simulink library "AEMS_Standard_Library"  (R2016b)
(part 5 of 39)

      |         else
      |             blocks_size = length(NewStatusstr);
      |             for r=length(NewStatusstr)+1:length(OldStatusstr)
      |                 lh = get_param([libb,'/Conversion_Subsystem_',num2str(r)],'Handle');
      |                 lc = get_param([libb,'/Data_Type_Conversion_',num2str(r)],'Handle');
      |                 l = get_param([libb,'/',OldStatusstr(r).Name],'Handle');
      |                 delete_block(lh);
      |                 delete_block(lc);
      |                 delete_block(l);
      |             end
      |             delete_line(find_system(libb,'FollowLinks','on','FindAll','on','LookUnderMasks','on','Type','line','Connected','off'));
      |         end
      |     end
      |     
      |     
      |     
      |     for i=1:count_DID
      |         n = num2str(i);
      |         if i==1
      |             tmp_sub = conv_subs;
      |             tmp_dataconv = data_converter;
      |             nameblk='Conversion_Subsystem';
      |         else
      |             tmp_sub = [conv_subs,'_',n];
      |             tmp_dataconv = [data_converter,'_',n];
      |             nameblk=['Conversion_Subsystem','_',n];
      |         end
      |         pos_i = get_param(tmp_sub,'Position');
      |         conv_type = get_param(tmp_sub,'MaskType');
      |         dc = get_param(tmp_dataconv,'Position');
      |         pos_i_o=pos_i;
      |         dc1 = dc;
      |         if length(upd_dmux.Outport)>=i
      |             r_upd_dmux = get(upd_dmux.Outport(i),'Position');
      |             pos_i_o(2)=r_upd_dmux(2)-(pos_i(4)-pos_i(2))/2;
      |             pos_i_o(4)=r_upd_dmux(2)+(pos_i(4)-pos_i(2))/2;
      |             dc1(2) = r_upd_dmux(2)-(dc(4)-dc(2))/2;
      |             dc1(4) = r_upd_dmux(2)+(dc(4)-dc(2))/2;
      |         end
      |         set_param(tmp_sub,'Position',pos_i_o);
      |         set_param(tmp_dataconv,'Position',dc1);
      |         
      |         ph_h = get_param(tmp_sub,'PortHandles');
      |         add_line(libb,ph_dmux.Outport(i),ph_h.Inport,'Autorouting','On');
      |         set_param(tmp_sub,'ShowName','off');
      |         set_param(tmp_dataconv,'ShowName','off');
      |         if ismember(NewStatusstr(i).DID_DataType,{'uint8','int8'}) && ~strcmp(conv_type,'AEMS_CONVERT_BYTE_TO_FLP')
      |             %If the ctrl reaches here means, this did is changed from Multibyte to 1 byte.
      |             replace_block(libb,'FollowLinks', 'on','Name',nameblk,'AEMS_Standard_Library/SUB/AEMS_CONVERT_BYTE_TO_FLP','noprompt');
      |         elseif ~ismember(NewStatusstr(i).DID_DataType,{'uint8','int8'}) && strcmp(conv_type,'AEMS_CONVERT_BYTE_TO_FLP')
      |             replace_block(libb,'FollowLinks', 'on','Name',nameblk,'AEMS_Standard_Library/SUB/AEMS_CONVERT_BUFFER_TO_FLP','noprompt');
      |         end
      |         set_param(tmp_sub,...
      |             'Resol',NewStatusstr(i).Resol,...
      |             'offset',NewStatusstr(i).Offset,...
      |             'DID_Datatype',NewStatusstr(i).DID_DataType);
      |         convertblk=get_param(tmp_sub,'LineHandles');
      |         datacovblk=get_param(tmp_dataconv,'LineHandles');
      |         dstblkhdl=get_param(datacovblk.Outport,'DstBlockHandle');
      |         if dstblkhdl==1
      |             ports_name = dstblkhdl;
      |         elseif dstblkhdl > 1
      |             if isequal(get_param(dstblkhdl(1),'BlockType'),'Outport')
      |                 ports_name = dstblkhdl(1);
      |             elseif isequal(get_param(dstblkhdl(2),'BlockType'),'Outport')
      |                 ports_name = dstblkhdl(2);
      |             end
      |         end
      |         
      |         set_param(ports_name,'Name',NewStatusstr(i).Name);
      |         pos_out_i = get_param(ports_name,'Position');
      |         
      |         pos_out_i_o=pos_out_i;
      |         pos_out_i_o(2)=(pos_i_o(2)+pos_i_o(4))/2-(pos_out_i(4)-pos_out_i(2))/2;
      |         pos_out_i_o(4)=(pos_i_o(2)+pos_i_o(4))/2+(pos_out_i(4)-pos_out_i(2))/2;
      |         set_param(dstblkhdl(1),'Position',pos_out_i_o);
      |     end
      | end
      | for i=1:blocks_size
      |     if i==1
      |         conv_blk_name = [libb,'/Conversion_Subsystem'];
      |     else
      |         conv_blk_name = [libb,'/Conversion_Subsystem_',num2str(i)];
      |     end
      |     if ~isequal(NewStatusstr(i).DID_DataType,OldStatusstr(i).DID_DataType)
      |         name_blk = get_param(conv_blk_name,'Name');
      |         if ismember(NewStatusstr(i).DID_DataType,{'uint8','int8'}) && ~ismember(OldStatusstr(i).DID_DataType,{'uint8','int8'})
      |             replace_block(libb,'FollowLinks', 'on','Name',name_blk,'AEMS_Standard_Library/SUB/AEMS_CONVERT_BYTE_TO_FLP','noprompt');
      |         elseif ~ismember(NewStatusstr(i).DID_DataType,{'uint8','int8'}) && ismember(OldStatusstr(i).DID_DataType,{'uint8','int8'})
      |             replace_block(libb,'FollowLinks', 'on','Name',name_blk,'AEMS_Standard_Library/SUB/AEMS_CONVERT_BUFFER_TO_FLP','noprompt');
      |         end
      |         set_param(conv_blk_name,'DID_Datatype',NewStatusstr(i).DID_DataType);
      |     end
      |     if ~isequal(NewStatusstr(i).Resol,OldStatusstr(i).Resol)
      |         set_param(conv_blk_name,'Resol',NewStatusstr(i).Resol);
      |     end
      |     if ~isequal(NewStatusstr(i).Offset,OldStatusstr(i).Offset)
      |         set_param(conv_blk_name,'offset',NewStatusstr(i).Offset);
      |     end
      |     if ~isequal(NewStatusstr(i).Name,OldStatusstr(i).Name)&& ~chg_status
      |         set(ou{i},'Name',NewStatusstr(i).Name);
      |     end
      | end
      | txtvisibility='%<MaskType> \n ConfigManagement : %<ConfigManagement> \n DID Abstract: %<DIDAbstract> \n Number of DID Variables: %<NumDIDVar>';
      | for i=1:count_DID
      |     n = num2str(i);
      |     txtvisibility=[txtvisibility,'\n %<OutVarName_',n,'> : {Resol = %<ResolDID_',n,'>, Offset = %<OffsetDID_',n,'>, DID_Monitoring_DataType = %<DataType_DID_',n,'>}'];
      | end
      | % wrfly_old = find_system(libh,'FollowLinks','on','LookunderMasks','all','MaskType','AEMS_NVM_WRITEONFLY');
      | % wrfly_new = get(libh,'NVMChecked');
      | % N_Inports=get_param(libb,'NumDIDVar');
      | % if strcmp(wrfly_new,'off')
      | %     if ~isempty(wrfly_old)
      | %         lh_wr = get_param(wr_fly,'LineHandles');
      | %         for hdl_len = 1:length(lh_wr.Inport)
      | %             if lh_wr.Inport(hdl_len)>0
      | %                 delete_line(lh_wr.Inport(hdl_len));
      | %             end
      | %         end
      | %         delete_line(lh_wr.Enable);
      | %         delete_block(wr_fly);
      | %     end
      | %     txtvisibility=[txtvisibility,'\n NVM WriteOnFly Variables : %<NVMChecked>'];
      | % else
      | %     if isempty(wrfly_old)
      | %         call_sub = get_param([libb,'/Callback_Subsystem'],'Position');
      | %         wrf_hand = add_block('AEMS_Standard_Library/MEM/AEMS_NVM_WRITEONFLY',[libb,'/AEMS_NVM_WRITEONFLY'],...
      | %             'Position',[call_sub(1)-200 call_sub(4)+50 call_sub(1)+50 call_sub(4)+120],'ChId',get_param(libb,'Channel'),'TriggerType','Enable');
      | %         lh_wr = get_param(wrf_hand,'PortHandles');
      | %         lh_perm = get_param(perm_sub,'PortHandles');
      | %         add_line(libb,lh_perm.Outport,lh_wr.Enable,'Autorouting','On');
      | %     else
      | %         newnvmchannel=get_param(libb,'Channel');
      | %         oldnvmchannel=get_param(wrfly_old,'ChId');
      | %         if ~strcmpi(newnvmchannel,oldnvmchannel)
      | %             set_param(wrfly_old,'ChId',newnvmchannel);
      | %         end
      | %     end
      | %     if isempty(wrfly_old)|| chg_status
      | %         write_hdles = get_param([libb,'/AEMS_NVM_WRITEONFLY'],'LineHandles');
      | %         for hdl_len = 1:length(write_hdles.Inport)
      | %             if ~isequal(write_hdles.Inport(hdl_len),-1)
      | %                 delete_line(write_hdles.Inport(hdl_len));
      | %             end
      | %         end
      | %         set_param([libb,'/AEMS_NVM_WRITEONFLY'],'NumInputs',N_Inports);
      | %         write_port = get_param([libb,'/AEMS_NVM_WRITEONFLY'],'PortHandles');
      | %         for r=1:length(NewStatusstr)
      | %             if(r==1)
      | %                 conversion_hdl = get_param([libb,'/Data_Type_Conversion'],'PortHandles');
      | %             else
      | %                 conversion_hdl = get_param([libb,'/Data_Type_Conversion_',num2str(r)],'PortHandles');
      | %             end
      | %             add_line(libb,conversion_hdl.Outport,write_port.Inport(r),'Autorouting','On');
      | %         end
      | %     end
      | %     txtvisibility=[txtvisibility,'\n NVM WriteOnFly Variables : %<NVMChecked> \n WriteOnFly Channel : %<Channel>'];
      | % end
      | % if ~strcmp(txtvisibility,old_txtvisibility)
      | %     set(libh,'AttributesFormatString',txtvisibility);
      | % end
      settings: AttributesFormatString=%<MaskType> \n ConfigManagement : %<ConfigManagement> \n DID Abstract: %<DIDAbstract> \n Number of DID Variables: %<NumDIDVar>\n %<OutVarName_1> : {Resol = %<ResolDID_1>, Offset = %<OffsetDID_1>, DID_Monitoring_DataType = %<DataType_DID_1>}
      mask Help:
      | eval('path_lib=fileparts(which(''AEMS_Standard_Library''));');
      | doc_path = [path_lib '\help\AEMS_DCM_DID_WRITEDATA.pdf'];
      | eval('open(doc_path)')
      mask TypeOptions NumDIDVar: 1 | 2 | 3 | 4 | 5 | 6 | 7 | 8 | 9 | 10 | 11 | 12 | 13 | 14 | 15 | 16 | 17 | 18 | 19 | 20 | 21 | 22 | 23 | 24 | 25 | 26 | 27 | 28 | 29 | 30 | 31 | 32 | 33 | 34 | 35 | 36 | 37 | 38 | 39 | 40 | 41 | 42 | 43 | 44 | 45 | 46 | 47 | 48 | 49 | 50 | 51 | 52 | 53 | 54 | 55 | 56 | 57 | 58 | 59 | 60 | 61 | 62 | 63 | 64 | 65 | 66 | 67 | 68 | 69 | 70 | 71 | 72 | 73 | 74 | 75 | 76 | 77 | 78 | 79 | 80 | 81 | 82 | 83 | 84 | 85 | 86 | 87 | 88 | 89 | 90 | 91 | 92 | 93 | 94 | 95 | 96 | 97 | 98 | 99 | 100 | 101 | 102 | 103 | 104 | 105 | 106 | 107 | 108 | 109 | 110 | 111 | 112 | 113 | 114 | 115 | 116 | 117 | 118 | 119 | 120 | 121 | 122 | 123 | 124 | 125 | 126 | 127 | 128 | 129 | 130 | 131 | 132 | 133 | 134 | 135 | 136 | 137 | 138 | 139 | 140 | 141 | 142 | 143 | 144 | 145 | 146 | 147 | 148 | 149 | 150 | 151 | 152 | 153 | 154 | 155 | 156 | 157 | 158 | 159 | 160 | 161 | 162 | 163 | 164 | 165 | 166 | 167 | 168 | 169 | 170 | 171 | 172 | 173 | 174 | 175 | 176 | 177 | 178 | 179 | 180 | 181 | 182 | 183 | 184 | 185 | 186 | 187 | 188 | 189 | 190 | 191 | 192 | 193 | 194 | 195 | 196 | 197 | 198 | 199 | 200 | 201 | 202 | 203 | 204 | 205 | 206 | 207 | 208 | 209 | 210 | 211 | 212 | 213 | 214 | 215 | 216 | 217 | 218 | 219 | 220 | 221 | 222 | 223 | 224 | 225 | 226 | 227 | 228 | 229 | 230 | 231 | 232 | 233 | 234 | 235 | 236 | 237 | 238 | 239 | 240 | 241 | 242 | 243 | 244 | 245 | 246 | 247 | 248 | 249 | 250 | 251 | 252 | 253 | 254 | 255 | 256 | 257 | 258 | 259 | 260 | 261 | 262 | 263 | 264 | 265 | 266 | 267 | 268 | 269 | 270 | 271 | 272 | 273 | 274 | 275 | 276 | 277 | 278 | 279 | 280 | 281 | 282 | 283 | 284 | 285 | 286 | 287 | 288 | 289 | 290 | 291 | 292 | 293 | 294 | 295 | 296 | 297 | 298 | 299 | 300 | 301 | 302 | 303 | 304 | 305 | 306 | 307 | 308 | 309 | 310 | 311 | 312 | 313 | 314 | 315 | 316 | 317 | 318 | 319 | 320 | 321 | 322 | 323 | 324 | 325 | 326 | 327 | 328 | 329 | 330 | 331 | 332 | 333 | 334 | 335 | 336 | 337 | 338 | 339 | 340 | 341 | 342 | 343 | 344 | 345 | 346 | 347 | 348 | 349 | 350 | 351 | 352 | 353 | 354 | 355 | 356 | 357 | 358 | 359 | 360 | 361 | 362 | 363 | 364 | 365 | 366 | 367 | 368 | 369 | 370 | 371 | 372 | 373 | 374 | 375 | 376 | 377 | 378 | 379 | 380 | 381 | 382 | 383 | 384 | 385 | 386 | 387 | 388 | 389 | 390 | 391 | 392 | 393 | 394 | 395 | 396 | 397 | 398 | 399 | 400
      mask Callback NumDIDVar:
      | DCM_WR_DATA_NumDIDVar = str2double(get(gcbh,'NumDIDVar'));
      | maskobj = Simulink.Mask.get(gcbh);
      | maskobj_old = maskobj.getDialogControls();
      | DCM_WR_DATA_second = maskobj_old.DialogControls(2);
      | show_hide_DID = DCM_WR_DATA_second.DialogControls;
      | 
      | for DID_j=2:length(show_hide_DID)
      |     show_hide_DID(DID_j).Visible = 'off';
      | end
      | 
      | for DID_j=DCM_WR_DATA_NumDIDVar+1:-1:2
      |     show_hide_DID(DID_j).Visible = 'on';
      | end
      | 
      | clear DCM_WR_DATA_NumDIDVar;
      | clear show_hide_DID;
      | clear maskobj;
      | clear maskobj_old;
      | clear DID_j;
      | clear DCM_WR_DATA_second;
      mask TypeOptions DataType_DID_1: int8 | uint8 | int16 | uint16 | int32 | uint32
      mask TypeOptions DataType_DID_2: int8 | uint8 | int16 | uint16 | int32 | uint32
      mask TypeOptions DataType_DID_3: int8 | uint8 | int16 | uint16 | int32 | uint32
      mask TypeOptions DataType_DID_4: int8 | uint8 | int16 | uint16 | int32 | uint32
      mask TypeOptions DataType_DID_5: int8 | uint8 | int16 | uint16 | int32 | uint32
      mask TypeOptions DataType_DID_6: int8 | uint8 | int16 | uint16 | int32 | uint32
      mask TypeOptions DataType_DID_7: int8 | uint8 | int16 | uint16 | int32 | uint32
      mask TypeOptions DataType_DID_8: int8 | uint8 | int16 | uint16 | int32 | uint32
      mask TypeOptions DataType_DID_9: int8 | uint8 | int16 | uint16 | int32 | uint32
      mask TypeOptions DataType_DID_10: int8 | uint8 | int16 | uint16 | int32 | uint32
      mask TypeOptions DataType_DID_11: int8 | uint8 | int16 | uint16 | int32 | uint32
      mask TypeOptions DataType_DID_12: int8 | uint8 | int16 | uint16 | int32 | uint32
      mask TypeOptions DataType_DID_13: int8 | uint8 | int16 | uint16 | int32 | uint32
      mask TypeOptions DataType_DID_14: int8 | uint8 | int16 | uint16 | int32 | uint32
      mask TypeOptions DataType_DID_15: int8 | uint8 | int16 | uint16 | int32 | uint32
      mask TypeOptions DataType_DID_16: int8 | uint8 | int16 | uint16 | int32 | uint32
      mask TypeOptions DataType_DID_17: int8 | uint8 | int16 | uint16 | int32 | uint32
      mask TypeOptions DataType_DID_18: int8 | uint8 | int16 | uint16 | int32 | uint32
      mask TypeOptions DataType_DID_19: int8 | uint8 | int16 | uint16 | int32 | uint32
      mask TypeOptions DataType_DID_20: int8 | uint8 | int16 | uint16 | int32 | uint32
      mask TypeOptions DataType_DID_21: int8 | uint8 | int16 | uint16 | int32 | uint32
      mask TypeOptions DataType_DID_22: int8 | uint8 | int16 | uint16 | int32 | uint32
      mask TypeOptions DataType_DID_23: int8 | uint8 | int16 | uint16 | int32 | uint32
      mask TypeOptions DataType_DID_24: int8 | uint8 | int16 | uint16 | int32 | uint32
      mask TypeOptions DataType_DID_25: int8 | uint8 | int16 | uint16 | int32 | uint32
      mask TypeOptions DataType_DID_26: int8 | uint8 | int16 | uint16 | int32 | uint32
      mask TypeOptions DataType_DID_27: int8 | uint8 | int16 | uint16 | int32 | uint32
      mask TypeOptions DataType_DID_28: int8 | uint8 | int16 | uint16 | int32 | uint32
      mask TypeOptions DataType_DID_29: int8 | uint8 | int16 | uint16 | int32 | uint32
      mask TypeOptions DataType_DID_30: int8 | uint8 | int16 | uint16 | int32 | uint32
      mask TypeOptions DataType_DID_31: int8 | uint8 | int16 | uint16 | int32 | uint32
      mask TypeOptions DataType_DID_32: int8 | uint8 | int16 | uint16 | int32 | uint32
      mask TypeOptions DataType_DID_33: int8 | uint8 | int16 | uint16 | int32 | uint32
      mask TypeOptions DataType_DID_34: int8 | uint8 | int16 | uint16 | int32 | uint32
      mask TypeOptions DataType_DID_35: int8 | uint8 | int16 | uint16 | int32 | uint32
      mask TypeOptions DataType_DID_36: int8 | uint8 | int16 | uint16 | int32 | uint32
      mask TypeOptions DataType_DID_37: int8 | uint8 | int16 | uint16 | int32 | uint32
      mask TypeOptions DataType_DID_38: int8 | uint8 | int16 | uint16 | int32 | uint32
      mask TypeOptions DataType_DID_39: int8 | uint8 | int16 | uint16 | int32 | uint32
      mask TypeOptions DataType_DID_40: int8 | uint8 | int16 | uint16 | int32 | uint32
      mask TypeOptions DataType_DID_41: int8 | uint8 | int16 | uint16 | int32 | uint32
      mask TypeOptions DataType_DID_42: int8 | uint8 | int16 | uint16 | int32 | uint32
      mask TypeOptions DataType_DID_43: int8 | uint8 | int16 | uint16 | int32 | uint32
      mask TypeOptions DataType_DID_44: int8 | uint8 | int16 | uint16 | int32 | uint32
      mask TypeOptions DataType_DID_45: int8 | uint8 | int16 | uint16 | int32 | uint32
      mask TypeOptions DataType_DID_46: int8 | uint8 | int16 | uint16 | int32 | uint32
      mask TypeOptions DataType_DID_47: int8 | uint8 | int16 | uint16 | int32 | uint32
      mask TypeOptions DataType_DID_48: int8 | uint8 | int16 | uint16 | int32 | uint32
      mask TypeOptions DataType_DID_49: int8 | uint8 | int16 | uint16 | int32 | uint32
      mask TypeOptions DataType_DID_50: int8 | uint8 | int16 | uint16 | int32 | uint32
      mask TypeOptions DataType_DID_51: int8 | uint8 | int16 | uint16 | int32 | uint32
      mask TypeOptions DataType_DID_52: int8 | uint8 | int16 | uint16 | int32 | uint32
      mask TypeOptions DataType_DID_53: int8 | uint8 | int16 | uint16 | int32 | uint32
      mask TypeOptions DataType_DID_54: int8 | uint8 | int16 | uint16 | int32 | uint32
      mask TypeOptions DataType_DID_55: int8 | uint8 | int16 | uint16 | int32 | uint32
      mask TypeOptions DataType_DID_56: int8 | uint8 | int16 | uint16 | int32 | uint32
      mask TypeOptions DataType_DID_57: int8 | uint8 | int16 | uint16 | int32 | uint32
      mask TypeOptions DataType_DID_58: int8 | uint8 | int16 | uint16 | int32 | uint32
      mask TypeOptions DataType_DID_59: int8 | uint8 | int16 | uint16 | int32 | uint32
      mask TypeOptions DataType_DID_60: int8 | uint8 | int16 | uint16 | int32 | uint32
      mask TypeOptions DataType_DID_61: int8 | uint8 | int16 | uint16 | int32 | uint32
      mask TypeOptions DataType_DID_62: int8 | uint8 | int16 | uint16 | int32 | uint32
      mask TypeOptions DataType_DID_63: int8 | uint8 | int16 | uint16 | int32 | uint32
      mask TypeOptions DataType_DID_64: int8 | uint8 | int16 | uint16 | int32 | uint32
      mask TypeOptions DataType_DID_65: int8 | uint8 | int16 | uint16 | int32 | uint32
      mask TypeOptions DataType_DID_66: int8 | uint8 | int16 | uint16 | int32 | uint32
      mask TypeOptions DataType_DID_67: int8 | uint8 | int16 | uint16 | int32 | uint32
      mask TypeOptions DataType_DID_68: int8 | uint8 | int16 | uint16 | int32 | uint32
      mask TypeOptions DataType_DID_69: int8 | uint8 | int16 | uint16 | int32 | uint32
      mask TypeOptions DataType_DID_70: int8 | uint8 | int16 | uint16 | int32 | uint32
      mask TypeOptions DataType_DID_71: int8 | uint8 | int16 | uint16 | int32 | uint32
      mask TypeOptions DataType_DID_72: int8 | uint8 | int16 | uint16 | int32 | uint32
      mask TypeOptions DataType_DID_73: int8 | uint8 | int16 | uint16 | int32 | uint32
      mask TypeOptions DataType_DID_74: int8 | uint8 | int16 | uint16 | int32 | uint32
      mask TypeOptions DataType_DID_75: int8 | uint8 | int16 | uint16 | int32 | uint32
      mask TypeOptions DataType_DID_76: int8 | uint8 | int16 | uint16 | int32 | uint32
      mask TypeOptions DataType_DID_77: int8 | uint8 | int16 | uint16 | int32 | uint32
      mask TypeOptions DataType_DID_78: int8 | uint8 | int16 | uint16 | int32 | uint32
      mask TypeOptions DataType_DID_79: int8 | uint8 | int16 | uint16 | int32 | uint32
      mask TypeOptions DataType_DID_80: int8 | uint8 | int16 | uint16 | int32 | uint32
      mask TypeOptions DataType_DID_81: int8 | uint8 | int16 | uint16 | int32 | uint32
      mask TypeOptions DataType_DID_82: int8 | uint8 | int16 | uint16 | int32 | uint32
      mask TypeOptions DataType_DID_83: int8 | uint8 | int16 | uint16 | int32 | uint32
      mask TypeOptions DataType_DID_84: int8 | uint8 | int16 | uint16 | int32 | uint32
      mask TypeOptions DataType_DID_85: int8 | uint8 | int16 | uint16 | int32 | uint32
      mask TypeOptions DataType_DID_86: int8 | uint8 | int16 | uint16 | int32 | uint32
      mask TypeOptions DataType_DID_87: int8 | uint8 | int16 | uint16 | int32 | uint32
      mask TypeOptions DataType_DID_88: int8 | uint8 | int16 | uint16 | int32 | uint32
      mask TypeOptions DataType_DID_89: int8 | uint8 | int16 | uint16 | int32 | uint32
      mask TypeOptions DataType_DID_90: int8 | uint8 | int16 | uint16 | int32 | uint32
      mask TypeOptions DataType_DID_91: int8 | uint8 | int16 | uint16 | int32 | uint32
      mask TypeOptions DataType_DID_92: int8 | uint8 | int16 | uint16 | int32 | uint32
      mask TypeOptions DataType_DID_93: int8 | uint8 | int16 | uint16 | int32 | uint32
      mask TypeOptions DataType_DID_94: int8 | uint8 | int16 | uint16 | int32 | uint32
      mask TypeOptions DataType_DID_95: int8 | uint8 | int16 | uint16 | int32 | uint32
      mask TypeOptions DataType_DID_96: int8 | uint8 | int16 | uint16 | int32 | uint32
      mask TypeOptions DataType_DID_97: int8 | uint8 | int16 | uint16 | int32 | uint32
      mask TypeOptions DataType_DID_98: int8 | uint8 | int16 | uint16 | int32 | uint32
      mask TypeOptions DataType_DID_99: int8 | uint8 | int16 | uint16 | int32 | uint32
      mask TypeOptions DataType_DID_100: int8 | uint8 | int16 | uint16 | int32 | uint32
      mask TypeOptions DataType_DID_101: int8 | uint8 | int16 | uint16 | int32 | uint32
      mask TypeOptions DataType_DID_102: int8 | uint8 | int16 | uint16 | int32 | uint32
      mask TypeOptions DataType_DID_103: int8 | uint8 | int16 | uint16 | int32 | uint32
      mask TypeOptions DataType_DID_104: int8 | uint8 | int16 | uint16 | int32 | uint32
      mask TypeOptions DataType_DID_105: int8 | uint8 | int16 | uint16 | int32 | uint32
      mask TypeOptions DataType_DID_106: int8 | uint8 | int16 | uint16 | int32 | uint32
      mask TypeOptions DataType_DID_107: int8 | uint8 | int16 | uint16 | int32 | uint32
      mask TypeOptions DataType_DID_108: int8 | uint8 | int16 | uint16 | int32 | uint32
      mask TypeOptions DataType_DID_109: int8 | uint8 | int16 | uint16 | int32 | uint32
      mask TypeOptions DataType_DID_110: int8 | uint8 | int16 | uint16 | int32 | uint32
      mask TypeOptions DataType_DID_111: int8 | uint8 | int16 | uint16 | int32 | uint32
      mask TypeOptions DataType_DID_112: int8 | uint8 | int16 | uint16 | int32 | uint32
      mask TypeOptions DataType_DID_113: int8 | uint8 | int16 | uint16 | int32 | uint32
      mask TypeOptions DataType_DID_114: int8 | uint8 | int16 | uint16 | int32 | uint32
      mask TypeOptions DataType_DID_115: int8 | uint8 | int16 | uint16 | int32 | uint32
      mask TypeOptions DataType_DID_116: int8 | uint8 | int16 | uint16 | int32 | uint32
      mask TypeOptions DataType_DID_117: int8 | uint8 | int16 | uint16 | int32 | uint32
      mask TypeOptions DataType_DID_118: int8 | uint8 | int16 | uint16 | int32 | uint32
      mask TypeOptions DataType_DID_119: int8 | uint8 | int16 | uint16 | int32 | uint32
      mask TypeOptions DataType_DID_120: int8 | uint8 | int16 | uint16 | int32 | uint32
      mask TypeOptions DataType_DID_121: int8 | uint8 | int16 | uint16 | int32 | uint32
      mask TypeOptions DataType_DID_122: int8 | uint8 | int16 | uint16 | int32 | uint32
      mask TypeOptions DataType_DID_123: int8 | uint8 | int16 | uint16 | int32 | uint32
      mask TypeOptions DataType_DID_124: int8 | uint8 | int16 | uint16 | int32 | uint32
      mask TypeOptions DataType_DID_125: int8 | uint8 | int16 | uint16 | int32 | uint32
      mask TypeOptions DataType_DID_126: int8 | uint8 | int16 | uint16 | int32 | uint32
      mask TypeOptions DataType_DID_127: int8 | uint8 | int16 | uint16 | int32 | uint32
      mask TypeOptions DataType_DID_128: int8 | uint8 | int16 | uint16 | int32 | uint32
      mask TypeOptions DataType_DID_129: int8 | uint8 | int16 | uint16 | int32 | uint32
      mask TypeOptions DataType_DID_130: int8 | uint8 | int16 | uint16 | int32 | uint32
      mask TypeOptions DataType_DID_131: int8 | uint8 | int16 | uint16 | int32 | uint32
      mask TypeOptions DataType_DID_132: int8 | uint8 | int16 | uint16 | int32 | uint32
      mask TypeOptions DataType_DID_133: int8 | uint8 | int16 | uint16 | int32 | uint32
      mask TypeOptions DataType_DID_134: int8 | uint8 | int16 | uint16 | int32 | uint32
      mask TypeOptions DataType_DID_135: int8 | uint8 | int16 | uint16 | int32 | uint32
      mask TypeOptions DataType_DID_136: int8 | uint8 | int16 | uint16 | int32 | uint32
      mask TypeOptions DataType_DID_137: int8 | uint8 | int16 | uint16 | int32 | uint32
      mask TypeOptions DataType_DID_138: int8 | uint8 | int16 | uint16 | int32 | uint32
      mask TypeOptions DataType_DID_139: int8 | uint8 | int16 | uint16 | int32 | uint32
      mask TypeOptions DataType_DID_140: int8 | uint8 | int16 | uint16 | int32 | uint32
      mask TypeOptions DataType_DID_141: int8 | uint8 | int16 | uint16 | int32 | uint32
      mask TypeOptions DataType_DID_142: int8 | uint8 | int16 | uint16 | int32 | uint32
      mask TypeOptions DataType_DID_143: int8 | uint8 | int16 | uint16 | int32 | uint32
      mask TypeOptions DataType_DID_144: int8 | uint8 | int16 | uint16 | int32 | uint32
      mask TypeOptions DataType_DID_145: int8 | uint8 | int16 | uint16 | int32 | uint32
      mask TypeOptions DataType_DID_146: int8 | uint8 | int16 | uint16 | int32 | uint32
      mask TypeOptions DataType_DID_147: int8 | uint8 | int16 | uint16 | int32 | uint32
      mask TypeOptions DataType_DID_148: int8 | uint8 | int16 | uint16 | int32 | uint32
      mask TypeOptions DataType_DID_149: int8 | uint8 | int16 | uint16 | int32 | uint32
      mask TypeOptions DataType_DID_150: int8 | uint8 | int16 | uint16 | int32 | uint32
      mask TypeOptions DataType_DID_151: int8 | uint8 | int16 | uint16 | int32 | uint32
      mask TypeOptions DataType_DID_152: int8 | uint8 | int16 | uint16 | int32 | uint32
      mask TypeOptions DataType_DID_153: int8 | uint8 | int16 | uint16 | int32 | uint32
      mask TypeOptions DataType_DID_154: int8 | uint8 | int16 | uint16 | int32 | uint32
      mask TypeOptions DataType_DID_155: int8 | uint8 | int16 | uint16 | int32 | uint32
      mask TypeOptions DataType_DID_156: int8 | uint8 | int16 | uint16 | int32 | uint32
      mask TypeOptions DataType_DID_157: int8 | uint8 | int16 | uint16 | int32 | uint32
      mask TypeOptions DataType_DID_158: int8 | uint8 | int16 | uint16 | int32 | uint32
      mask TypeOptions DataType_DID_159: int8 | uint8 | int16 | uint16 | int32 | uint32
      mask TypeOptions DataType_DID_160: int8 | uint8 | int16 | uint16 | int32 | uint32
      mask TypeOptions DataType_DID_161: int8 | uint8 | int16 | uint16 | int32 | uint32
      mask TypeOptions DataType_DID_162: int8 | uint8 | int16 | uint16 | int32 | uint32
      mask TypeOptions DataType_DID_163: int8 | uint8 | int16 | uint16 | int32 | uint32
      mask TypeOptions DataType_DID_164: int8 | uint8 | int16 | uint16 | int32 | uint32
      mask TypeOptions DataType_DID_165: int8 | uint8 | int16 | uint16 | int32 | uint32
      mask TypeOptions DataType_DID_166: int8 | uint8 | int16 | uint16 | int32 | uint32
      mask TypeOptions DataType_DID_167: int8 | uint8 | int16 | uint16 | int32 | uint32
      mask TypeOptions DataType_DID_168: int8 | uint8 | int16 | uint16 | int32 | uint32
      mask TypeOptions DataType_DID_169: int8 | uint8 | int16 | uint16 | int32 | uint32
      mask TypeOptions DataType_DID_170: int8 | uint8 | int16 | uint16 | int32 | uint32
      mask TypeOptions DataType_DID_171: int8 | uint8 | int16 | uint16 | int32 | uint32
      mask TypeOptions DataType_DID_172: int8 | uint8 | int16 | uint16 | int32 | uint32
      mask TypeOptions DataType_DID_173: int8 | uint8 | int16 | uint16 | int32 | uint32
      mask TypeOptions DataType_DID_174: int8 | uint8 | int16 | uint16 | int32 | uint32
      mask TypeOptions DataType_DID_175: int8 | uint8 | int16 | uint16 | int32 | uint32
      mask TypeOptions DataType_DID_176: int8 | uint8 | int16 | uint16 | int32 | uint32
      mask TypeOptions DataType_DID_177: int8 | uint8 | int16 | uint16 | int32 | uint32
      mask TypeOptions DataType_DID_178: int8 | uint8 | int16 | uint16 | int32 | uint32
      mask TypeOptions DataType_DID_179: int8 | uint8 | int16 | uint16 | int32 | uint32
      mask TypeOptions DataType_DID_180: int8 | uint8 | int16 | uint16 | int32 | uint32
      mask TypeOptions DataType_DID_181: int8 | uint8 | int16 | uint16 | int32 | uint32
      mask TypeOptions DataType_DID_182: int8 | uint8 | int16 | uint16 | int32 | uint32
      mask TypeOptions DataType_DID_183: int8 | uint8 | int16 | uint16 | int32 | uint32
      mask TypeOptions DataType_DID_184: int8 | uint8 | int16 | uint16 | int32 | uint32
      mask TypeOptions DataType_DID_185: int8 | uint8 | int16 | uint16 | int32 | uint32
      mask TypeOptions DataType_DID_186: int8 | uint8 | int16 | uint16 | int32 | uint32
      mask TypeOptions DataType_DID_187: int8 | uint8 | int16 | uint16 | int32 | uint32
      mask TypeOptions DataType_DID_188: int8 | uint8 | int16 | uint16 | int32 | uint32
      mask TypeOptions DataType_DID_189: int8 | uint8 | int16 | uint16 | int32 | uint32
      mask TypeOptions DataType_DID_190: int8 | uint8 | int16 | uint16 | int32 | uint32
      mask TypeOptions DataType_DID_191: int8 | uint8 | int16 | uint16 | int32 | uint32
      mask TypeOptions DataType_DID_192: int8 | uint8 | int16 | uint16 | int32 | uint32
      mask TypeOptions DataType_DID_193: int8 | uint8 | int16 | uint16 | int32 | uint32
      mask TypeOptions DataType_DID_194: int8 | uint8 | int16 | uint16 | int32 | uint32
      mask TypeOptions DataType_DID_195: int8 | uint8 | int16 | uint16 | int32 | uint32
      mask TypeOptions DataType_DID_196: int8 | uint8 | int16 | uint16 | int32 | uint32
      mask TypeOptions DataType_DID_197: int8 | uint8 | int16 | uint16 | int32 | uint32
      mask TypeOptions DataType_DID_198: int8 | uint8 | int16 | uint16 | int32 | uint32
      mask TypeOptions DataType_DID_199: int8 | uint8 | int16 | uint16 | int32 | uint32
      mask TypeOptions DataType_DID_200: int8 | uint8 | int16 | uint16 | int32 | uint32
      mask TypeOptions DataType_DID_201: int8 | uint8 | int16 | uint16 | int32 | uint32
      mask TypeOptions DataType_DID_202: int8 | uint8 | int16 | uint16 | int32 | uint32
      mask TypeOptions DataType_DID_203: int8 | uint8 | int16 | uint16 | int32 | uint32
      mask TypeOptions DataType_DID_204: int8 | uint8 | int16 | uint16 | int32 | uint32
      mask TypeOptions DataType_DID_205: int8 | uint8 | int16 | uint16 | int32 | uint32
      mask TypeOptions DataType_DID_206: int8 | uint8 | int16 | uint16 | int32 | uint32
      mask TypeOptions DataType_DID_207: int8 | uint8 | int16 | uint16 | int32 | uint32
      mask TypeOptions DataType_DID_208: int8 | uint8 | int16 | uint16 | int32 | uint32
      mask TypeOptions DataType_DID_209: int8 | uint8 | int16 | uint16 | int32 | uint32
      mask TypeOptions DataType_DID_210: int8 | uint8 | int16 | uint16 | int32 | uint32
      mask TypeOptions DataType_DID_211: int8 | uint8 | int16 | uint16 | int32 | uint32
      mask TypeOptions DataType_DID_212: int8 | uint8 | int16 | uint16 | int32 | uint32
      mask TypeOptions DataType_DID_213: int8 | uint8 | int16 | uint16 | int32 | uint32
      mask TypeOptions DataType_DID_214: int8 | uint8 | int16 | uint16 | int32 | uint32
      mask TypeOptions DataType_DID_215: int8 | uint8 | int16 | uint16 | int32 | uint32
      mask TypeOptions DataType_DID_216: int8 | uint8 | int16 | uint16 | int32 | uint32
      mask TypeOptions DataType_DID_217: int8 | uint8 | int16 | uint16 | int32 | uint32
      mask TypeOptions DataType_DID_218: int8 | uint8 | int16 | uint16 | int32 | uint32
      mask TypeOptions DataType_DID_219: int8 | uint8 | int16 | uint16 | int32 | uint32
      mask TypeOptions DataType_DID_220: int8 | uint8 | int16 | uint16 | int32 | uint32
      mask TypeOptions DataType_DID_221: int8 | uint8 | int16 | uint16 | int32 | uint32
      mask TypeOptions DataType_DID_222: int8 | uint8 | int16 | uint16 | int32 | uint32
      mask TypeOptions DataType_DID_223: int8 | uint8 | int16 | uint16 | int32 | uint32
      mask TypeOptions DataType_DID_224: int8 | uint8 | int16 | uint16 | int32 | uint32
      mask TypeOptions DataType_DID_225: int8 | uint8 | int16 | uint16 | int32 | uint32
      mask TypeOptions DataType_DID_226: int8 | uint8 | int16 | uint16 | int32 | uint32
      mask TypeOptions DataType_DID_227: int8 | uint8 | int16 | uint16 | int32 | uint32
      mask TypeOptions DataType_DID_228: int8 | uint8 | int16 | uint16 | int32 | uint32
      mask TypeOptions DataType_DID_229: int8 | uint8 | int16 | uint16 | int32 | uint32
      mask TypeOptions DataType_DID_230: int8 | uint8 | int16 | uint16 | int32 | uint32
      mask TypeOptions DataType_DID_231: int8 | uint8 | int16 | uint16 | int32 | uint32
      mask TypeOptions DataType_DID_232: int8 | uint8 | int16 | uint16 | int32 | uint32
      mask TypeOptions DataType_DID_233: int8 | uint8 | int16 | uint16 | int32 | uint32
      mask TypeOptions DataType_DID_234: int8 | uint8 | int16 | uint16 | int32 | uint32
      mask TypeOptions DataType_DID_235: int8 | uint8 | int16 | uint16 | int32 | uint32
      mask TypeOptions DataType_DID_236: int8 | uint8 | int16 | uint16 | int32 | uint32
      mask TypeOptions DataType_DID_237: int8 | uint8 | int16 | uint16 | int32 | uint32
      mask TypeOptions DataType_DID_238: int8 | uint8 | int16 | uint16 | int32 | uint32
      mask TypeOptions DataType_DID_239: int8 | uint8 | int16 | uint16 | int32 | uint32
      mask TypeOptions DataType_DID_240: int8 | uint8 | int16 | uint16 | int32 | uint32
      mask TypeOptions DataType_DID_241: int8 | uint8 | int16 | uint16 | int32 | uint32
      mask TypeOptions DataType_DID_242: int8 | uint8 | int16 | uint16 | int32 | uint32
      mask TypeOptions DataType_DID_243: int8 | uint8 | int16 | uint16 | int32 | uint32
      mask TypeOptions DataType_DID_244: int8 | uint8 | int16 | uint16 | int32 | uint32
      mask TypeOptions DataType_DID_245: int8 | uint8 | int16 | uint16 | int32 | uint32
      mask TypeOptions DataType_DID_246: int8 | uint8 | int16 | uint16 | int32 | uint32
      mask TypeOptions DataType_DID_247: int8 | uint8 | int16 | uint16 | int32 | uint32
      mask TypeOptions DataType_DID_248: int8 | uint8 | int16 | uint16 | int32 | uint32
      mask TypeOptions DataType_DID_249: int8 | uint8 | int16 | uint16 | int32 | uint32
      mask TypeOptions DataType_DID_250: int8 | uint8 | int16 | uint16 | int32 | uint32
      mask TypeOptions DataType_DID_251: int8 | uint8 | int16 | uint16 | int32 | uint32
      mask TypeOptions DataType_DID_252: int8 | uint8 | int16 | uint16 | int32 | uint32
      mask TypeOptions DataType_DID_253: int8 | uint8 | int16 | uint16 | int32 | uint32
      mask TypeOptions DataType_DID_254: int8 | uint8 | int16 | uint16 | int32 | uint32
      mask TypeOptions DataType_DID_255: int8 | uint8 | int16 | uint16 | int32 | uint32
      mask TypeOptions DataType_DID_256: int8 | uint8 | int16 | uint16 | int32 | uint32
      mask TypeOptions DataType_DID_257: int8 | uint8 | int16 | uint16 | int32 | uint32
      mask TypeOptions DataType_DID_258: int8 | uint8 | int16 | uint16 | int32 | uint32
      mask TypeOptions DataType_DID_259: int8 | uint8 | int16 | uint16 | int32 | uint32
      mask TypeOptions DataType_DID_260: int8 | uint8 | int16 | uint16 | int32 | uint32
      mask TypeOptions DataType_DID_261: int8 | uint8 | int16 | uint16 | int32 | uint32
      mask TypeOptions DataType_DID_262: int8 | uint8 | int16 | uint16 | int32 | uint32
      mask TypeOptions DataType_DID_263: int8 | uint8 | int16 | uint16 | int32 | uint32
      mask TypeOptions DataType_DID_264: int8 | uint8 | int16 | uint16 | int32 | uint32
      mask TypeOptions DataType_DID_265: int8 | uint8 | int16 | uint16 | int32 | uint32
      mask TypeOptions DataType_DID_266: int8 | uint8 | int16 | uint16 | int32 | uint32
      mask TypeOptions DataType_DID_267: int8 | uint8 | int16 | uint16 | int32 | uint32
      mask TypeOptions DataType_DID_268: int8 | uint8 | int16 | uint16 | int32 | uint32
      mask TypeOptions DataType_DID_269: int8 | uint8 | int16 | uint16 | int32 | uint32
      mask TypeOptions DataType_DID_270: int8 | uint8 | int16 | uint16 | int32 | uint32
      mask TypeOptions DataType_DID_271: int8 | uint8 | int16 | uint16 | int32 | uint32
      mask TypeOptions DataType_DID_272: int8 | uint8 | int16 | uint16 | int32 | uint32
      mask TypeOptions DataType_DID_273: int8 | uint8 | int16 | uint16 | int32 | uint32
      mask TypeOptions DataType_DID_274: int8 | uint8 | int16 | uint16 | int32 | uint32
      mask TypeOptions DataType_DID_275: int8 | uint8 | int16 | uint16 | int32 | uint32
      mask TypeOptions DataType_DID_276: int8 | uint8 | int16 | uint16 | int32 | uint32
      mask TypeOptions DataType_DID_277: int8 | uint8 | int16 | uint16 | int32 | uint32
      mask TypeOptions DataType_DID_278: int8 | uint8 | int16 | uint16 | int32 | uint32
      mask TypeOptions DataType_DID_279: int8 | uint8 | int16 | uint16 | int32 | uint32
      mask TypeOptions DataType_DID_280: int8 | uint8 | int16 | uint16 | int32 | uint32
      mask TypeOptions DataType_DID_281: int8 | uint8 | int16 | uint16 | int32 | uint32
      mask TypeOptions DataType_DID_282: int8 | uint8 | int16 | uint16 | int32 | uint32
      mask TypeOptions DataType_DID_283: int8 | uint8 | int16 | uint16 | int32 | uint32
      mask TypeOptions DataType_DID_284: int8 | uint8 | int16 | uint16 | int32 | uint32
      mask TypeOptions DataType_DID_285: int8 | uint8 | int16 | uint16 | int32 | uint32
      mask TypeOptions DataType_DID_286: int8 | uint8 | int16 | uint16 | int32 | uint32
      mask TypeOptions DataType_DID_287: int8 | uint8 | int16 | uint16 | int32 | uint32
      mask TypeOptions DataType_DID_288: int8 | uint8 | int16 | uint16 | int32 | uint32
      mask TypeOptions DataType_DID_289: int8 | uint8 | int16 | uint16 | int32 | uint32
      mask TypeOptions DataType_DID_290: int8 | uint8 | int16 | uint16 | int32 | uint32
      mask TypeOptions DataType_DID_291: int8 | uint8 | int16 | uint16 | int32 | uint32
      mask TypeOptions DataType_DID_292: int8 | uint8 | int16 | uint16 | int32 | uint32
      mask TypeOptions DataType_DID_293: int8 | uint8 | int16 | uint16 | int32 | uint32
      mask TypeOptions DataType_DID_294: int8 | uint8 | int16 | uint16 | int32 | uint32
      mask TypeOptions DataType_DID_295: int8 | uint8 | int16 | uint16 | int32 | uint32
      mask TypeOptions DataType_DID_296: int8 | uint8 | int16 | uint16 | int32 | uint32
      mask TypeOptions DataType_DID_297: int8 | uint8 | int16 | uint16 | int32 | uint32
      mask TypeOptions DataType_DID_298: int8 | uint8 | int16 | uint16 | int32 | uint32
      mask TypeOptions DataType_DID_299: int8 | uint8 | int16 | uint16 | int32 | uint32
      mask TypeOptions DataType_DID_300: int8 | uint8 | int16 | uint16 | int32 | uint32
      mask TypeOptions DataType_DID_301: int8 | uint8 | int16 | uint16 | int32 | uint32
      mask TypeOptions DataType_DID_302: int8 | uint8 | int16 | uint16 | int32 | uint32
      mask TypeOptions DataType_DID_303: int8 | uint8 | int16 | uint16 | int32 | uint32
      mask TypeOptions DataType_DID_304: int8 | uint8 | int16 | uint16 | int32 | uint32
      mask TypeOptions DataType_DID_305: int8 | uint8 | int16 | uint16 | int32 | uint32
      mask TypeOptions DataType_DID_306: int8 | uint8 | int16 | uint16 | int32 | uint32
      mask TypeOptions DataType_DID_307: int8 | uint8 | int16 | uint16 | int32 | uint32
      mask TypeOptions DataType_DID_308: int8 | uint8 | int16 | uint16 | int32 | uint32
      mask TypeOptions DataType_DID_309: int8 | uint8 | int16 | uint16 | int32 | uint32
      mask TypeOptions DataType_DID_310: int8 | uint8 | int16 | uint16 | int32 | uint32
      mask TypeOptions DataType_DID_311: int8 | uint8 | int16 | uint16 | int32 | uint32
      mask TypeOptions DataType_DID_312: int8 | uint8 | int16 | uint16 | int32 | uint32
      mask TypeOptions DataType_DID_313: int8 | uint8 | int16 | uint16 | int32 | uint32
      mask TypeOptions DataType_DID_314: int8 | uint8 | int16 | uint16 | int32 | uint32
      mask TypeOptions DataType_DID_315: int8 | uint8 | int16 | uint16 | int32 | uint32
      mask TypeOptions DataType_DID_316: int8 | uint8 | int16 | uint16 | int32 | uint32
      mask TypeOptions DataType_DID_317: int8 | uint8 | int16 | uint16 | int32 | uint32
      mask TypeOptions DataType_DID_318: int8 | uint8 | int16 | uint16 | int32 | uint32
      mask TypeOptions DataType_DID_319: int8 | uint8 | int16 | uint16 | int32 | uint32
      mask TypeOptions DataType_DID_320: int8 | uint8 | int16 | uint16 | int32 | uint32
      mask TypeOptions DataType_DID_321: int8 | uint8 | int16 | uint16 | int32 | uint32
      mask TypeOptions DataType_DID_322: int8 | uint8 | int16 | uint16 | int32 | uint32
      mask TypeOptions DataType_DID_323: int8 | uint8 | int16 | uint16 | int32 | uint32
      mask TypeOptions DataType_DID_324: int8 | uint8 | int16 | uint16 | int32 | uint32
      mask TypeOptions DataType_DID_325: int8 | uint8 | int16 | uint16 | int32 | uint32
      mask TypeOptions DataType_DID_326: int8 | uint8 | int16 | uint16 | int32 | uint32
      mask TypeOptions DataType_DID_327: int8 | uint8 | int16 | uint16 | int32 | uint32
      mask TypeOptions DataType_DID_328: int8 | uint8 | int16 | uint16 | int32 | uint32
      mask TypeOptions DataType_DID_329: int8 | uint8 | int16 | uint16 | int32 | uint32
      mask TypeOptions DataType_DID_330: int8 | uint8 | int16 | uint16 | int32 | uint32
      mask TypeOptions DataType_DID_331: int8 | uint8 | int16 | uint16 | int32 | uint32
      mask TypeOptions DataType_DID_332: int8 | uint8 | int16 | uint16 | int32 | uint32
      mask TypeOptions DataType_DID_333: int8 | uint8 | int16 | uint16 | int32 | uint32
      mask TypeOptions DataType_DID_334: int8 | uint8 | int16 | uint16 | int32 | uint32
      mask TypeOptions DataType_DID_335: int8 | uint8 | int16 | uint16 | int32 | uint32
      mask TypeOptions DataType_DID_336: int8 | uint8 | int16 | uint16 | int32 | uint32
      mask TypeOptions DataType_DID_337: int8 | uint8 | int16 | uint16 | int32 | uint32
      mask TypeOptions DataType_DID_338: int8 | uint8 | int16 | uint16 | int32 | uint32
      mask TypeOptions DataType_DID_339: int8 | uint8 | int16 | uint16 | int32 | uint32
      mask TypeOptions DataType_DID_340: int8 | uint8 | int16 | uint16 | int32 | uint32
      mask TypeOptions DataType_DID_341: int8 | uint8 | int16 | uint16 | int32 | uint32
      mask TypeOptions DataType_DID_342: int8 | uint8 | int16 | uint16 | int32 | uint32
      mask TypeOptions DataType_DID_343: int8 | uint8 | int16 | uint16 | int32 | uint32
      mask TypeOptions DataType_DID_344: int8 | uint8 | int16 | uint16 | int32 | uint32
      mask TypeOptions DataType_DID_345: int8 | uint8 | int16 | uint16 | int32 | uint32
      mask TypeOptions DataType_DID_346: int8 | uint8 | int16 | uint16 | int32 | uint32
      mask TypeOptions DataType_DID_347: int8 | uint8 | int16 | uint16 | int32 | uint32
      mask TypeOptions DataType_DID_348: int8 | uint8 | int16 | uint16 | int32 | uint32
      mask TypeOptions DataType_DID_349: int8 | uint8 | int16 | uint16 | int32 | uint32
      mask TypeOptions DataType_DID_350: int8 | uint8 | int16 | uint16 | int32 | uint32
      mask TypeOptions DataType_DID_351: int8 | uint8 | int16 | uint16 | int32 | uint32
      mask TypeOptions DataType_DID_352: int8 | uint8 | int16 | uint16 | int32 | uint32
      mask TypeOptions DataType_DID_353: int8 | uint8 | int16 | uint16 | int32 | uint32
      mask TypeOptions DataType_DID_354: int8 | uint8 | int16 | uint16 | int32 | uint32
      mask TypeOptions DataType_DID_355: int8 | uint8 | int16 | uint16 | int32 | uint32
      mask TypeOptions DataType_DID_356: int8 | uint8 | int16 | uint16 | int32 | uint32
      mask TypeOptions DataType_DID_357: int8 | uint8 | int16 | uint16 | int32 | uint32
      mask TypeOptions DataType_DID_358: int8 | uint8 | int16 | uint16 | int32 | uint32
      mask TypeOptions DataType_DID_359: int8 | uint8 | int16 | uint16 | int32 | uint32
      mask TypeOptions DataType_DID_360: int8 | uint8 | int16 | uint16 | int32 | uint32
      mask TypeOptions DataType_DID_361: int8 | uint8 | int16 | uint16 | int32 | uint32
      mask TypeOptions DataType_DID_362: int8 | uint8 | int16 | uint16 | int32 | uint32
      mask TypeOptions DataType_DID_363: int8 | uint8 | int16 | uint16 | int32 | uint32
      mask TypeOptions DataType_DID_364: int8 | uint8 | int16 | uint16 | int32 | uint32
      mask TypeOptions DataType_DID_365: int8 | uint8 | int16 | uint16 | int32 | uint32
      mask TypeOptions DataType_DID_366: int8 | uint8 | int16 | uint16 | int32 | uint32
      mask TypeOptions DataType_DID_367: int8 | uint8 | int16 | uint16 | int32 | uint32
      mask TypeOptions DataType_DID_368: int8 | uint8 | int16 | uint16 | int32 | uint32
      mask TypeOptions DataType_DID_369: int8 | uint8 | int16 | uint16 | int32 | uint32
      mask TypeOptions DataType_DID_370: int8 | uint8 | int16 | uint16 | int32 | uint32
      mask TypeOptions DataType_DID_371: int8 | uint8 | int16 | uint16 | int32 | uint32
      mask TypeOptions DataType_DID_372: int8 | uint8 | int16 | uint16 | int32 | uint32
      mask TypeOptions DataType_DID_373: int8 | uint8 | int16 | uint16 | int32 | uint32
      mask TypeOptions DataType_DID_374: int8 | uint8 | int16 | uint16 | int32 | uint32
      mask TypeOptions DataType_DID_375: int8 | uint8 | int16 | uint16 | int32 | uint32
      mask TypeOptions DataType_DID_376: int8 | uint8 | int16 | uint16 | int32 | uint32
      mask TypeOptions DataType_DID_377: int8 | uint8 | int16 | uint16 | int32 | uint32
      mask TypeOptions DataType_DID_378: int8 | uint8 | int16 | uint16 | int32 | uint32
      mask TypeOptions DataType_DID_379: int8 | uint8 | int16 | uint16 | int32 | uint32
      mask TypeOptions DataType_DID_380: int8 | uint8 | int16 | uint16 | int32 | uint32
      mask TypeOptions DataType_DID_381: int8 | uint8 | int16 | uint16 | int32 | uint32
      mask TypeOptions DataType_DID_382: int8 | uint8 | int16 | uint16 | int32 | uint32
      mask TypeOptions DataType_DID_383: int8 | uint8 | int16 | uint16 | int32 | uint32
      mask TypeOptions DataType_DID_384: int8 | uint8 | int16 | uint16 | int32 | uint32
      mask TypeOptions DataType_DID_385: int8 | uint8 | int16 | uint16 | int32 | uint32
      mask TypeOptions DataType_DID_386: int8 | uint8 | int16 | uint16 | int32 | uint32
      mask TypeOptions DataType_DID_387: int8 | uint8 | int16 | uint16 | int32 | uint32
      mask TypeOptions DataType_DID_388: int8 | uint8 | int16 | uint16 | int32 | uint32
      mask TypeOptions DataType_DID_389: int8 | uint8 | int16 | uint16 | int32 | uint32
      mask TypeOptions DataType_DID_390: int8 | uint8 | int16 | uint16 | int32 | uint32
      mask TypeOptions DataType_DID_391: int8 | uint8 | int16 | uint16 | int32 | uint32
      mask TypeOptions DataType_DID_392: int8 | uint8 | int16 | uint16 | int32 | uint32
      mask TypeOptions DataType_DID_393: int8 | uint8 | int16 | uint16 | int32 | uint32
      mask TypeOptions DataType_DID_394: int8 | uint8 | int16 | uint16 | int32 | uint32
      mask TypeOptions DataType_DID_395: int8 | uint8 | int16 | uint16 | int32 | uint32
      mask TypeOptions DataType_DID_396: int8 | uint8 | int16 | uint16 | int32 | uint32
      mask TypeOptions DataType_DID_397: int8 | uint8 | int16 | uint16 | int32 | uint32
      mask TypeOptions DataType_DID_398: int8 | uint8 | int16 | uint16 | int32 | uint32
      mask TypeOptions DataType_DID_399: int8 | uint8 | int16 | uint16 | int32 | uint32
      mask TypeOptions DataType_DID_400: int8 | uint8 | int16 | uint16 | int32 | uint32
      mask Display:
      | blk_handle = gcbh;
      | try
      |     set(blk_handle,'MaskIconOpaque','transparent');
      | catch
      |     set(blk_handle,'MaskIconOpaque','off');
      | end
  AEMS_DCM_GETDATA : Subsystem  Tag=[LIB]  mask(AEMS_DCM_GETDATA){GetdataAbstract=DCM_GETDATA, NumOutputs=2, OutputName1=Val_1, OutputName2=Val_2, OutputName3=Val_3, OutputName4=Val_4, OutputName5=Val_5, OutputName6=Val_6, OutputName7=Val_7, OutputName8=Val_8, OutputName9=Val_9, OutputName10=Val_10, OutputName11=Val_11, OutputName12=Val_12, OutputName13=Val_13, OutputName14=Val_14, OutputName15=Val_15, OutputName16=Val_16, OutputName17=Val_17, OutputName18=Val_18, OutputName19=Val_19, OutputName20=Val_20, OutputName21=Val_21, OutputName22=Val_22, OutputName23=Val_23, OutputName24=Val_24, OutputName25=Val_25, OutputName26=Val_26, OutputName27=Val_27, OutputName28=Val_28, OutputName29=Val_29, OutputName30=Val_30, OutputName31=Val_31, OutputName32=Val_32, OutputName33=Val_33, OutputName34=Val_34, OutputName35=Val_35, OutputName36=Val_36, OutputName37=Val_37, OutputName38=Val_38, OutputName39=Val_39, OutputName40=Val_40, OutputName41=Val_41, OutputName42=Val_42, OutputName43=Val_43, OutputName44=Val_44, OutputName45=Val_45, OutputName46=Val_46, OutputName47=Val_47, OutputName48=Val_48, OutputName49=Val_49, OutputName50=Val_50, OutputName51=Val_51, OutputName52=Val_52, OutputName53=Val_53, OutputName54=Val_54, OutputName55=Val_55, OutputName56=Val_56, OutputName57=Val_57, OutputName58=Val_58, OutputName59=Val_59, OutputName60=Val_60, OutputName61=Val_61, OutputName62=Val_62, OutputName63=Val_63, OutputName64=Val_64}
      mask prompts: GetdataAbstract "Getdata Abstract"; NumOutputs "Number of Outputs"; OutputName1 "Output Name 1"; OutputName2 "Output Name 2"; OutputName3 "Output Name 3"; OutputName4 "Output Name 4"; OutputName5 "Output Name 5"; OutputName6 "Output Name 6"; OutputName7 "Output Name 7"; OutputName8 "Output Name 8"; OutputName9 "Output Name 9"; OutputName10 "Output Name 10"; OutputName11 "Output Name 11"; OutputName12 "Output Name 12"; OutputName13 "Output Name 13"; OutputName14 "Output Name 14"; OutputName15 "Output Name 15"; OutputName16 "Output Name 16"; OutputName17 "Output Name 17"; OutputName18 "Output Name 18"; OutputName19 "Output Name 19"; OutputName20 "Output Name 20"; OutputName21 "Output Name 21"; OutputName22 "Output Name 22"; OutputName23 "Output Name 23"; OutputName24 "Output Name 24"; OutputName25 "Output Name 25"; OutputName26 "Output Name 26"; OutputName27 "Output Name 27"; OutputName28 "Output Name 28"; OutputName29 "Output Name 29"; OutputName30 "Output Name 30"; OutputName31 "Output Name 31"; OutputName32 "Output Name 32"; OutputName33 "Output Name 33"; OutputName34 "Output Name 34"; OutputName35 "Output Name 35"; OutputName36 "Output Name 36"; OutputName37 "Output Name 37"; OutputName38 "Output Name 38"; OutputName39 "Output Name 39"; OutputName40 "Output Name 40"; OutputName41 "Output Name 41"; OutputName42 "Output Name 42"; OutputName43 "Output Name 43"; OutputName44 "Output Name 44"; OutputName45 "Output Name 45"; OutputName46 "Output Name 46"; OutputName47 "Output Name 47"; OutputName48 "Output Name 48"; OutputName49 "Output Name 49"; OutputName50 "Output Name 50"; OutputName51 "Output Name 51"; OutputName52 "Output Name 52"; OutputName53 "Output Name 53"; OutputName54 "Output Name 54"; OutputName55 "Output Name 55"; OutputName56 "Output Name 56"; OutputName57 "Output Name 57"; OutputName58 "Output Name 58"; OutputName59 "Output Name 59"; OutputName60 "Output Name 60"; OutputName61 "Output Name 61"; OutputName62 "Output Name 62"; OutputName63 "Output Name 63"; OutputName64 "Output Name 64"
      mask help:
      | The block create the Outports depends on the mask parameters value (Number of Outputs and Outports name which are given in the mask parameter)
      | Reference to AUTOSAR specification:
      | - AUTOSAR Service Name:  Dcm_GetVin (Ref. [SWS_Dcm_00950])
      |
      | -PARAMETERS-
      | Getdata Abstract = Dcm_GetVin
      | Number of Output variables = Number of Outputs
      mask init:
      | ThisBlk = gcb;
      | Demux_Blk_Path = [ThisBlk,'/Demux'];
      | Demux_Blk_Pos  = get_param(Demux_Blk_Path,'Position');
      | 
      | OutPort_Blocks = find_system(ThisBlk,'LookUnderMasks','all','FollowLinks','on','SearchDepth',1,'BlockType','Outport');
      | Conv_Blocks = find_system(ThisBlk,'FollowLinks','on','LookunderMasks','all','regexp','on','BlockType','DataTypeConversion','Name','^Convblock_');
      | Num_Of_Outport_Blks = numel(OutPort_Blocks);
      | 
      | %Get Current OutPort_String.
      |   OutportNames_From_OutportBlocks = get_param(OutPort_Blocks,'Name'); %#ok<NASGU>
      |   OutportNames_From_MaskParams = {};%Initialize with emby cell, 
      |  for cnt=1:NumOutputs
      |       OutportNames_From_MaskParams{end+1} = get_param(ThisBlk,['OutputName',num2str(cnt)]);       %#ok<NASGU>
      |  end
      |  
      | %Error check:
      | Uniq_OutportNames_From_MaskParams = unique(OutportNames_From_MaskParams);
      | if numel(Uniq_OutportNames_From_MaskParams)~=numel(OutportNames_From_MaskParams)
      |     %If the ctrl reaches here means, some of the names are repeated. So
      |     %throw error.
      |     errordlg('Some of the names are repeated. Please verify');
      |     return;
      | end
      |  
      | if(Num_Of_Outport_Blks == NumOutputs) && isequal(OutportNames_From_MaskParams,OutportNames_From_OutportBlocks')
      |     
      |    % the number of outport blocks and NumOutputs are same and outport names
      |    % from mask parameter and from outport blocks are same control will
      |    % reach here
      |    %Do nothing.
      |     
      | else 
      |     
      |     
      |     
      |     % STEP 1 :FIrst delete all the existing outports & lines
      |     delete_block(OutPort_Blocks);
      |     
      |     for i=1:length(Conv_Blocks)
      |         conv_PH = get_param(Conv_Blocks{i},'PortHandles');
      |         LineHandles = get(conv_PH.Outport,'Line');
      |         if numel(conv_PH.Outport)==1
      |             % In this case there is only one outport, so LineHandles wil be a
      |             % single data. It's not a cell arry.
      |             try
      |                 delete(LineHandles);
      |             end
      |         else
      |             %In this case there r multiple outports, LineHandles will b a cell
      |             %arrry. so handle it using "{:}".
      |             try
      |                 delete(LineHandles{:});
      |             end
      |         end        
      |     end
      |     delete_block(Conv_Blocks);
      |     % STEP 2 : delete all the unconnected lines
      |     %Inside Masked subsytem, "find_system()" wont work to get the unconnected lines
      |     % So handle them using PortHandles. I'm sure there will be valid
      |     % no.of.OUtports so  I dont' cross check for 0 or Invalid port counts.
      |     % I call delete function blindly.
      |     Demux_PH = get_param(Demux_Blk_Path,'PortHandles');
      |     LineHandles = get(Demux_PH.Outport,'Line');
      |     if numel(Demux_PH.Outport)==1
      |         % In this case there is only one outport, so LineHandles wil be a
      |         % single data. It's not a cell arry.
      |         try
      |             delete(LineHandles);
      |         end
      |     else
      |         %In this case there r multiple outports, LineHandles will b a cell
      |         %arrry. so handle it using "{:}".
      |         try
      |             delete(LineHandles{:});
      |         end
      |     end
      |     
      |     %STEP 3  % Set the position of Demux blk as per no.of.ports..
      |     %Demux_Blk_Pos
      |     Height_Of_DemuxBlk = 10 + (NumOutputs *30);
      |     %WHile framing the new positon of the demux block, just determine the
      |     %Y2 Position don't disturbe X1,Y1,X2 postions.
      |     Demux_Blk_Pos(4)      = Demux_Blk_Pos(2) + Height_Of_DemuxBlk;
      |     set_param(Demux_Blk_Path,'Outputs',num2str(NumOutputs),'Position',Demux_Blk_Pos);
      |     PH_Demx = get_param(Demux_Blk_Path,'PortHandles');
      |     %STEP 4  % Add OUtport blocks & Connect it to Demux.
      |        %STEP 4  % Add OUtport blocks & Connect it to Demux.     
      |     for PortIdx = 1:NumOutputs        
      |         OutportName     = OutportNames_From_MaskParams{PortIdx};
      |         Demuxs_This_PortPosition = get(PH_Demx.Outport(PortIdx),'Position');
      |         
      |         ConvPosition(1) = Demuxs_This_PortPosition(1)+100;
      |         ConvPosition(3) = Demuxs_This_PortPosition(1)+150;
      |         ConvPosition(2) = Demuxs_This_PortPosition(2)-15;
      |         ConvPosition(4) = Demuxs_This_PortPosition(2)+15;
      |         
      |         OutportPosition(1) = Demuxs_This_PortPosition(1)+200;
      |         OutportPosition(3) = Demuxs_This_PortPosition(1)+230;
      |         OutportPosition(2) = Demuxs_This_PortPosition(2)-7;
      |         OutportPosition(4) = Demuxs_This_PortPosition(2)+7;
      |         OutportBlkPath  = [ThisBlk,'/',OutportName];
      |         ConvName=['Convblock_',OutportName];
      |         ConvBlkPath  = [ThisBlk,'/',ConvName];
      |         add_block('built-in/DataTypeConversion',ConvBlkPath,'Position',ConvPosition,'ShowName','off');
      |         add_line(ThisBlk,['Demux/',num2str(PortIdx)],[ConvName,'/1'],'autorouting','on');
      |         
      |         add_block('built-in/Outport',OutportBlkPath,'Position',OutportPosition,'Backgroundcolor','Orange');
      |         add_line(ThisBlk,[ConvName,'/1'],[OutportName,'/1'],'autorouting','on');
      |     end
      |     Attribute_Format_String_Part1 = '%<MaskType> \n Getdata Abstract : %<GetdataAbstract> \n Number of Outputs: %<NumOutputs>';
      |     Attribute_Format_String_Part2 = '';
      |     for Idx=1:NumOutputs
      |         Attribute_Format_String_Part2 = [Attribute_Format_String_Part2,'\n Output Name ', num2str(Idx),' : %<OutputName',num2str(Idx),'>'];
      |     end       
      |     Attribute_Format_String = [Attribute_Format_String_Part1,Attribute_Format_String_Part2];    
      |     set_param(ThisBlk,'AttributesFormatString',Attribute_Format_String);
      |     
      |     %Set position of the Ground, DTC blocks inside.    
      |     Demx_Inport_Position = get(PH_Demx.Inport,'Position');
      |     DTC_Blk_Path = [ThisBlk,'/Data Type Conversion1'];
      |     DTC_Blk_Pos  = get_param(DTC_Blk_Path,'Position');
      |     DTC_Blk_Pos(2) = Demx_Inport_Position(2)-10;
      |     DTC_Blk_Pos(4) = Demx_Inport_Position(2)+10;
      |     set_param(DTC_Blk_Path,'Position',DTC_Blk_Pos);
      |     
      |     GrnBlk_Path   = [ThisBlk,'/Ground'];
      |     GrnBlk_Pos    = get_param(GrnBlk_Path,'Position');
      |     GrnBlk_Pos(2) = DTC_Blk_Pos(2);
      |     GrnBlk_Pos(4) = DTC_Blk_Pos(4);
      |     set_param(GrnBlk_Path,'Position',GrnBlk_Pos);
      | 
      | end
      settings: AttributesFormatString=%<MaskType> \n Getdata Abstract : %<GetdataAbstract> \n Number of Outputs: %<NumOutputs>\n Output Name 1 : %<OutputName1>\n Output Name 2 : %<OutputName2>
      mask Help:
      | eval('path_lib=fileparts(which(''AEMS_Standard_Library''));');
      | mskblk=get_param(gcbh,'MaskType');
      | doc_path = [path_lib '\Help\',mskblk,'.pdf'];
      | eval('open(doc_path)');
      mask TypeOptions NumOutputs: 1 | 2 | 3 | 4 | 5 | 6 | 7 | 8 | 9 | 10 | 11 | 12 | 13 | 14 | 15 | 16 | 17 | 18 | 19 | 20 | 21 | 22 | 23 | 24 | 25 | 26 | 27 | 28 | 29 | 30 | 31 | 32 | 33 | 34 | 35 | 36 | 37 | 38 | 39 | 40 | 41 | 42 | 43 | 44 | 45 | 46 | 47 | 48 | 49 | 50 | 51 | 52 | 53 | 54 | 55 | 56 | 57 | 58 | 59 | 60 | 61 | 62 | 63 | 64
      mask Callback NumOutputs:
      | ThisBlk = gcb;
      |     Outputs_From_get_param = get_param(ThisBlk,'NumOutputs');%Why using get_param(), y not the direct name 'NumOutputs', Bcos Itsn't b updated @ this place.
      |     Outputs_From_get_param = str2double(Outputs_From_get_param);
      |     MaskString_Part1 = cell(1,2+Outputs_From_get_param);%why 2 +NumOutputs ? Bcos these many fields will b visible in the mask.
      |     MaskString_Part1(:) = {'on'};
      |     MaskString_Part2    = cell(1,66-numel(MaskString_Part1));%Why 66? Bcos there r 66 mask params in total. Among them "2+NumOutputs" will b visible other won't
      |     MaskString_Part2(:) = {'off'};
      |     MaskString = [MaskString_Part1,MaskString_Part2];
      |     set_param(ThisBlk,'MaskVisibilities',MaskString);
  AEMS_DCM_GETPROGCONDITIONS : Subsystem  Tag=[LIB]  mask(AEMS_DCM_GETPROGCONDITIONS){}
      mask help:
      | This library calls AUTOSAR standard functions.
      | To know more details, please refer AUTOSAR [SWS_Dcm_00544].
      settings: AttributesFormatString=%<MaskType>
      mask Display: disp(['Dcm_GetProgConditions']);
  AEMS_DCM_GETSESCTRLTYPE : Subsystem  Tag=[LIB]  mask(AEMS_DCM_GETSESCTRLTYPE){}
      mask help:
      | This function provides the active session control type value.
      | Reference to AUTOSAR specification:
      | - AUTOSAR Service Name:  Dcm_GetSesCtrlType (Ref. [SWS_Dcm_00339])
      |
      |
      | SesCtrlType : Active Session Control Type value Content is according to "diagnosticSessionType" parameter of DiagnosticSessionControl request
      |
      | Std_ReturnType : E_OK: this value is always returned.
      settings: AttributesFormatString=%<MaskType>
      mask Help:
      | eval('path_lib=fileparts(which(''AEMS_Standard_Library''));');
      | mskblk=get_param(gcbh,'MaskType');
      | doc_path = [path_lib '\Help\',mskblk,'.pdf'];
      | eval('open(doc_path)');
      mask Display: disp('AEMS_DCM_GETSESCTRLTYPE\n');
  AEMS_DCM_IO_RETURN_CONTROL_TO_ECU : Subsystem  Tag=[LIB]  mask(AEMS_DCM_IO_RETURN_CONTROL_TO_ECU){DIDAbstract=DCM_IO_XXXX}
      mask prompts: DIDAbstract "DID Abstract"
      mask help:
      | This function requests to the application to return control to ECU of an IOControl.
      |
      | It generate Request Write from DCM tools to set DID Variable by value of DCM tools. Request Write changes from FALSE to TRUE and inversely whenever it is called.
      |
      | - AUTOSAR Service Name:  Xxx_ReturnControlToECU (Ref. [SWS_Dcm_01285])
      |
      | -OUTPUTS-
      | Flag_Req_RtCtrToECU: Request to return control to ECU of an IOControl
      mask init:
      | hh = gcbh;
      | DIDAbstractstr=get_param(hh,'DIDAbstract'); 
      | Callbkstr=strcat('DataServices_',strtrim(DIDAbstractstr),'_ReturnControlToECU');
      | namepo1=strcat('Flag_Req_RtCtrToECU_',DIDAbstractstr);
      settings: AttributesFormatString=|
      | %<MaskType>
      | DID Abstract : %<DIDAbstract>
      mask Help:
      | eval('path_lib=fileparts(which(''AEMS_Standard_Library''));');
      | mskblk=get_param(gcbh,'MaskType');
      | doc_path = [path_lib '\Help\',mskblk,'.pdf'];
      | eval('open(doc_path)');
      mask Display: port_label('output',1,namepo1);
  AEMS_DCM_IO_SHORT_TERM_ADJUSTMENT : Subsystem  Tag=[LIB]  mask(AEMS_DCM_IO_SHORT_TERM_ADJUSTMENT){DIDAbstract=DCM_IO_XXXX, configuration_management=0, Cxx_DID_xxxx_IO_min=Cxx_DID_xxxx_IO_min, Cxx_DID_xxxx_IO_max=Cxx_DID_xxxx_IO_max, DataType=uint8, Resol=1, offset=0}
      mask prompts: DIDAbstract "DID Abstract"; configuration_management "Configuration Management"; Cxx_DID_xxxx_IO_min "Minimum of IO signal"; Cxx_DID_xxxx_IO_max "Maximum of IO signal"; DataType "DID DataType"; Resol "Resolution of DID"; offset "Offset of DID"
      mask help:
      | This function requests to the application to adjust the IO signal
      | Reference to AUTOSAR specification:
      | - AUTOSAR Service Name:  Xxx_ShortTermAdjustment.
      | - Reference: [SWS_Dcm_00802]
      |
      | -INPUTS-
      | Generic_Conditions_RoutineIO: Generic condition
      | Specific_Conditions_IO_XXXX: Specific condition of DID Variable
      |
      | -PARAMETERS-
      | Configuration Management: Configuration Management (TRUE or FALSE)
      | Minimum of IO signal: Cxx_dcm_io_min_xxxx
      | Maximum of IO signal: Cxx_dcm_io_max_xxxx
      | DID Abstract: Abstract of DID pre-defined
      | Offset of DID Variable: 	Offset of DID Variable
      | Resolution of DID Variable: 	Resolution of DID Variable
      | Size of DID Variable: 	Byte Number of DID Variable
      mask init:
      | This_Blk = gcb;
      | Blk_handle = gcbh;
      | 
      | DIDAbstractstr=get_param(Blk_handle,'DIDAbstract');
      | Callbkstr=strcat('DataServices_',strtrim(DIDAbstractstr),'_ShortTermAdjustement');
      | Conv_Subsystem_Path = [This_Blk,'/Conversion_Subsystem/Conversion_Subsystem'];
      | Parent_Of_Conv_Subsystem = get_param(Conv_Subsystem_Path,'Parent');
      | MaskType_Of_Existing_Conv_Subsystem = get_param(Conv_Subsystem_Path,'MaskType');
      | BlockType_Of_Existing_Conv_Subsystem = get_param(Conv_Subsystem_Path,'BlockType');
      | 
      | %% Setting the mask label for inports and outports
      | namepi1='Generic_Conditions_IORoutine';
      | namepi2=strcat('Specific_Conditions_',DIDAbstractstr);
      | namepo1=strcat('Value_Write_',DIDAbstractstr);
      | namepo2=strcat('Flag_Request_',DIDAbstractstr);
      | 
      | %% Get the parameter values from the mask
      | Resol_of_DID=get_param(Blk_handle,'Resol');
      | Offset_of_DID=get_param(Blk_handle,'offset');
      | DID_Data_Type=get_param(Blk_handle,'DataType');
      | 
      | if ismember(DID_Data_Type,'boolean') % DID_Data_Type is 'boolean', then "Data Type Conversion" will be added
      |     Expected_Mask_Type_Of_Conv_SubSystem = 'DataTypeConversion';
      |     set_param([This_Blk,'/Conversion_Subsystem/Demux'],'Outputs','[1]');
      | elseif ismember(DID_Data_Type,{'uint8','int8'}) % DID_Data_Type is 'uint8/int8', then "AEMS_CONVERT_BYTE_TO_FLP" will be added
      |     Expected_Mask_Type_Of_Conv_SubSystem = 'AEMS_CONVERT_BYTE_TO_FLP';
      |     set_param([This_Blk,'/Conversion_Subsystem/Demux'],'Outputs','[1]');
      | elseif ismember(DID_Data_Type,{'uint16','int16'}) % DID_Data_Type is 'uint16/int16/uint32/int32', then "AEMS_CONVERT_BUFFER_TO_FLP" will be added
      |     Expected_Mask_Type_Of_Conv_SubSystem = 'AEMS_CONVERT_BUFFER_TO_FLP';
      |     set_param([This_Blk,'/Conversion_Subsystem/Demux'],'Outputs','[2]');
      | elseif ismember(DID_Data_Type,{'uint32','int32'}) % DID_Data_Type is 'uint16/int16/uint32/int32', then "AEMS_CONVERT_BUFFER_TO_FLP" will be added
      |     Expected_Mask_Type_Of_Conv_SubSystem = 'AEMS_CONVERT_BUFFER_TO_FLP';
      |     set_param([This_Blk,'/Conversion_Subsystem/Demux'],'Outputs','[4]');
      | end
      | 
      | %% Replace blocks according to the chosen DID_DataType
      | if strcmp(Expected_Mask_Type_Of_Conv_SubSystem,MaskType_Of_Existing_Conv_Subsystem) || strcmp(Expected_Mask_Type_Of_Conv_SubSystem,BlockType_Of_Existing_Conv_Subsystem)
      |     %do nothing
      | elseif strcmp(Expected_Mask_Type_Of_Conv_SubSystem,'AEMS_CONVERT_BYTE_TO_FLP')%Replace the block with "AEMS_CONVERT_BYTE_TO_FLP"
      |     replace_block(This_Blk,'FollowLinks','on','Parent',Parent_Of_Conv_Subsystem,'Name','Conversion_Subsystem','AEMS_Standard_Library/SUB/AEMS_CONVERT_BYTE_TO_FLP','noprompt');
      | elseif strcmp(Expected_Mask_Type_Of_Conv_SubSystem,'AEMS_CONVERT_BUFFER_TO_FLP') %Replace the block with "AEMS_CONVERT_BUFFER_TO_FLP"
      |     replace_block(This_Blk,'FollowLinks','on','Parent',Parent_Of_Conv_Subsystem,'Name','Conversion_Subsystem','AEMS_Standard_Library/SUB/AEMS_CONVERT_BUFFER_TO_FLP','noprompt');
      | else %Replace the block with "Data Type Conversion"
      |     convert_blk_hdl=replace_block(This_Blk,'FollowLinks','on','Parent',Parent_Of_Conv_Subsystem,'Name','Conversion_Subsystem','built-in/DataTypeConversion','noprompt');
      |     set_param(char(convert_blk_hdl),'OutDataTypeStr','Inherit: Inherit via back propagation','Showname','off');
      | end
      | 
      | %% Set the parameter values from the mask to the Conversion_Subsystem block
      | if ~isequal(DID_Data_Type,'boolean')
      |     set_param(Conv_Subsystem_Path,'Resol',Resol_of_DID);
      |     set_param(Conv_Subsystem_Path,'offset',Offset_of_DID);
      |     set_param(Conv_Subsystem_Path,'DID_Datatype',DID_Data_Type);
      | end
      settings: AttributesFormatString=|
      | %<MaskType>
      | DID Abstract : %<DIDAbstract>
      | Config. Management : %<configuration_management>
      | Min. IO Signals :  %<Cxx_DID_xxxx_IO_min>,  Max. IO Signals : %<Cxx_DID_xxxx_IO_max>
      | DID DataType : %<DataType>, Resol of DID: %<Resol>, Offset of DID: %<offset>
      mask Help:
      | eval('path_lib=fileparts(which(''AEMS_Standard_Library''));');
      | mskblk=get_param(gcbh,'MaskType');
      | doc_path = [path_lib '\Help\',mskblk,'.pdf'];
      | eval('open(doc_path)');
      mask TypeOptions DataType: boolean | int8 | uint8 | int16 | uint16 | int32 | uint32
      mask Display:
      | port_label('input',1,namepi1);
      | port_label('input',2,namepi2);
      | port_label('output',1,namepo1);
      | port_label('output',2,namepo2);
  AEMS_DCM_REQUEST_RESULT : Subsystem  Tag=[LIB]  mask(AEMS_DCM_REQUEST_RESULT){DIDAbstract=DCM_REQ_RESULT_XXXX, Routine_Type_xxxx=Routine_Type_xxxx}
      mask prompts: DIDAbstract "RID Abstract"; Routine_Type_xxxx "Routine Type"
      mask help:
      | This function requests to the application the result of a routine execution.
      | AUTOSAR Interface: Xxx_RequestResults (Ref. [SWS_Dcm_91013]).
      |
      | Std_ReturnType Xxx_RequestResults(DcmDspRoutineSignalType* dataOut_1,
      | Dcm_NegativeResponseCodeType* ErrorCode)
      |
      | dataOut_1, ErrorCode: terminated to represent return values to DCM Tools.
      |
      | -INPUTS-
      | Routine_xxxx_Status: Routine Status of XXXX RID
      |
      | -PARAMETERS-
      | RID Abstract: Abstract of RID
      | Routine Type: Routine Type (3 for Renault)
      mask init:
      | hh = gcbh;
      | DIDAbstractstr=get_param(hh,'DIDAbstract'); 
      | namepi1=strcat('Routine_',DIDAbstractstr,'_Status');
      settings: AttributesFormatString=|
      | %<MaskType>
      | RID Abstract: %<DIDAbstract>
      | Routine Type: %<Routine_Type_xxxx>
      mask Help:
      | eval('path_lib=fileparts(which(''AEMS_Standard_Library''));');
      | mskblk=get_param(gcbh,'MaskType');
      | doc_path = [path_lib '\Help\',mskblk,'.pdf'];
      | eval('open(doc_path)');
      mask Display: port_label('input',1,namepi1);
  AEMS_DCM_START_ROUTINE : Subsystem  Tag=[LIB]  mask(AEMS_DCM_START_ROUTINE){DIDAbstract=DCM_START_XXXX, Routine_Type_xxxx=3, Routine_Status_Running=Nnx_dcm_rt_run_stt, Routine_Status_Aborted=Nnx_dcm_rt_abrt_stt}
      mask prompts: DIDAbstract "RID Abstract"; Routine_Type_xxxx "Routine Type"; Routine_Status_Running "Enumerate: Routine Status Running"; Routine_Status_Aborted "Enumerate: Routine Status Aborted"
      mask help:
      | This function requests to the application to start the execution of a routine.
      | AUTOSAR Interface: Xxx_Start (Ref. [SWS_Dcm_01203])
      |
      | Std_ReturnType Xxx_Start(DcmDspRoutineSignalType dataOut_1,
      | Dcm_NegativeResponseCodeType ErrorCode)
      |
      | dataOut_1, ErrorCode: terminated to represent return values to DCM Tools.
      |
      | -INPUTS-
      | Generic_Conditions_Routine: Generic condition
      | Specific_Conditions_Routine_xxxx: Specific condition of XXXX RID
      | Routine_Status: Routine status
      | Routine_xxxx_Status: Routine status (Running, Disabled, Aborted, etc)
      |
      | -OUTPUTS-
      | Flag_request_xxxx_DCM: Flag request from START Routine
      |
      | -PARAMETERS-
      | RID Abstract: Abstract of RID
      | Routine Type: Routine Type (3 for Renault)
      | Routine Status Running: Routine Status Running (Nnx_dcm_rt_run_stt)
      | Routine Status Aborted: Routine Status Aborted (Nnx_dcm_rt_abrt_stt)
      mask init: same as AEMS_Standard_Library/DCM/AEMS_DCM_CONDITIONCHECKREAD
      settings: AttributesFormatString=|
      | %<MaskType>
      | RID Abstract: %<DIDAbstract>
      | Routine Type: %<Routine_Type_xxxx>
      | Routine Status Running: %<Routine_Status_Running>
      | Routine Status Aborted: %<Routine_Status_Aborted>
      mask Help:
      | eval('path_lib=fileparts(which(''AEMS_Standard_Library''));');
      | mskblk=get_param(gcbh,'MaskType');
      | doc_path = [path_lib '\Help\',mskblk,'.pdf'];
      | eval('open(doc_path)');
      mask Display:
      | port_label('input',1,namepi1);
      | port_label('input',2,namepi2);
      | port_label('input',3,namepi3);
      | port_label('input',4,namepi4);
      | port_label('output',1,namepo1);
  AEMS_DCM_STOP_ROUTINE : Subsystem  Tag=[LIB]  mask(AEMS_DCM_STOP_ROUTINE){DIDAbstract=DCM_STOP_XXXX, Routine_Type_xxxx=3, Routine_Status_Running=Nnx_dcm_rt_run_stt, Routine_Status_Aborted=Nnx_dcm_rt_abrt_stt}
      mask prompts: DIDAbstract "RID Abstract"; Routine_Type_xxxx "Routine Type"; Routine_Status_Running "Enumerate: Routine Status Running"; Routine_Status_Aborted "Enumerate: Routine Status Aborted"
      mask help:
      | This function requests to the application to stop the execution of a routine.
      | AUTOSAR Interface: Xxx_Stop (Ref. [SWS_Dcm_01204]).
      | Std_ReturnType Xxx_Stop(DcmDspRoutineSignalType dataOut_1,
      | Dcm_NegativeResponseCodeType* ErrorCode)
      |
      | dataOut_1, ErrorCode: terminated to represent return values to DCM Tools.
      |
      | -INPUTS-
      | Routine_xxxx_Status: Routine Status of XXXX RID
      |
      | -OUTPUTS-
      | Flag_request_XXXX_DCM_Stop: Flag request stop for XXXX RID
      |
      | -PARAMETERS-
      | RID Abstract: Abstract of RID
      | Routine Type: Routine Type (3 for Renault)
      | Routine_Status_Running: Routine Status Running (Nnx_dcm_rt_run_stt)
      | Routine_Status_Aborted: Routine Status Aborted (Nnx_dcm_rt_abrt_stt)
      mask init:
      | hh = gcbh;
      | DIDAbstractstr=get_param(hh,'DIDAbstract'); 
      | Callbkstr=strcat('DataServices_',strtrim(DIDAbstractstr),'_WriteData');
      | namepi1=strcat('Routine_',DIDAbstractstr,'_Status');
      | namepo1=strcat('Flag_Request_',DIDAbstractstr);
      settings: AttributesFormatString=|
      | %<MaskType>
      | RID Abstract = %<DIDAbstract>
      | Routine_Type = %<Routine_Type_xxxx>
      | Routine Status Running : %<Routine_Status_Running>
      | Routine Status Aborted : %<Routine_Status_Aborted>
      mask Help:
      | eval('path_lib=fileparts(which(''AEMS_Standard_Library''));');
      | mskblk=get_param(gcbh,'MaskType');
      | doc_path = [path_lib '\Help\',mskblk,'.pdf'];
      | eval('open(doc_path)');
      mask Display:
      | port_label('input',1,namepi1);
      | port_label('output',1,namepo1);
  AEMS_FLOAT_TO_FXP : Subsystem  Tag=[LIB]  mask(AEMS_FLOAT_TO_FXP){Resol=1, Offset=0, OutputFixedPointDatatype=uint8}
      mask prompts: Resol "Resolution (Physical)"; Offset "Offset (Physical)"
      mask help:
      | Takes a physical signal as input and outputs a physical data in fixed point.
      |
      |  - PHYS : Physical Value (ex. Vxx_msr_tq_req / vTWN).
      |  - FXP : Fixed point signal (ex. Vxx_pid_2ch ).
      mask init:
      | ThisBlk = gcb;
      | Bpath = [ThisBlk,'/OutputDatatype'];
      | OutputDatatype = get_param(gcb,'OutputFixedPointDatatype');
      | set_param(Bpath,'OutDataTypeStr',OutputDatatype);
      settings: AttributesFormatString=|
      | %<MaskType>
      | Resolution = %<Resol>
      | Offset = %<Offset>
      | Output Fixed Point Datatype=%<OutputFixedPointDatatype>
      mask Help:
      | eval('path_lib=fileparts(which(''AEMS_Standard_Library''));');
      | mskblk=get_param(gcbh,'MaskType');
      | doc_path = [path_lib '\help\',mskblk,'.pdf'];
      | eval('open(doc_path)');
      mask TypeOptions OutputFixedPointDatatype: uint8 | int8 | uint16 | int16 | uint32 | int32
      mask Display:
      | TofxpLib_mask = ['To FXP \n ' 'Resolution (Physical) = ' num2str(Resol) '\n Offset (Physical) =' num2str(Offset) ];
      | disp(TofxpLib_mask);
      | port_label('input',1,'phys')
      | port_label('output',1,'fxp')
      | plot([5,5,5])
      | plot([6,6,6])
  AEMS_FLOAT_TO_FXP_WITH_LIMIT : Subsystem  Tag=[LIB]  mask(AEMS_FLOAT_TO_FXP_WITH_LIMIT){Resol=0.5, Offset=0, Min=0, Max=120, OutputFixedPointDatatype=uint8}
      mask prompts: Resol "Resolution (Physical)"; Offset "Offset (Physical)"; Min "Minimum (Physical)"; Max "Maximum (Physical)"
      mask help:
      | Takes a physical signal (either floating point or fixed point) as input and output a physical signal data typed in fixed point.
      |
      |  - PHYS : Physical Value (ex. Vxx_msr_tq_req / vTWN).
      |  - FXP : Fixed point signal (ex. Vxx_pid_2ch ).
      mask init:
      | ThisBlk = gcb;
      | Bpath = [ThisBlk,'/OutputDatatype'];
      | OutputDatatype = get_param(gcb,'OutputFixedPointDatatype');
      | set_param(Bpath,'OutDataTypeStr',OutputDatatype);
      | 
      | Min_Hex = (Min-Offset)/Resol; %Hex value of Min
      | Max_Hex = (Max-Offset)/Resol; %Hex value of Max
      | 
      | %Initial Checks:
      | if (Min_Hex > Max_Hex )
      |     disp(Min_Hex);
      |     disp(Max_Hex);    
      |     error('Physical Min Value Should be less than the Physical Max value');
      | end
      | 
      | %Chk for min/max values
      | 
      | switch OutputDatatype
      |     
      |     case 'int8'
      |         Possible_Min_Hex = -128;
      |         Possible_Max_Hex = 127;
      |     case 'uint8'
      |         Possible_Min_Hex = 0;
      |         Possible_Max_Hex = 255;
      |     case 'int16'
      |         Possible_Min_Hex = -32768;
      |         Possible_Max_Hex = 32767;
      |     case 'uint16'
      |         Possible_Min_Hex = 0;
      |         Possible_Max_Hex = 65535;
      |     case 'int32'
      |         Possible_Min_Hex = -2147483648;
      |         Possible_Max_Hex = 2147483647;
      |     case 'uint32'
      |         Possible_Min_Hex = 0;
      |         Possible_Max_Hex = 4294967295;
      | 
      | end
      | 
      | if (Min_Hex < Possible_Min_Hex)
      |     %     msg = sprintf(['\n','For the resolution of "',num2str(Resol),'" and Offset of "',num2str(Offset),'",\n',...
      |     %         'and output dataThe Physical Max value "',num2str(Max) ,'" can''t fit in 2 byte']);
      |     msg = sprintf(['\n','The physical min "',num2str(Min),'" is invalid for the specified configuration,\n',...
      |         ' Resolution = "',num2str(Resol),'",Offset = "',num2str(Offset),'", OutputDataType "',OutputDatatype,'"']);
      |     error(msg); %#ok<SPERR>
      | elseif (Max_Hex > Possible_Max_Hex)
      |     msg = sprintf(['\n','The physical max "',num2str(Max),'" is invalid for the specified configuration,\n',...
      |         ' Resolution = "',num2str(Resol),'",Offset = "',num2str(Offset),'", OutputDataType "',OutputDatatype,'"']);
      |     error(msg); %#ok<SPERR>
      | end
      settings: AttributesFormatString=|
      | %<MaskType>
      | Resolution = %<Resol>
      | Offset = %<Offset>
      | Range = [%<Min>   %<Max>]
      | Output Fixed Point Datatype=%<OutputFixedPointDatatype>
      mask Help:
      | eval('path_lib=fileparts(which(''AEMS_Standard_Library''));');
      | mskblk=get_param(gcbh,'MaskType');
      | doc_path = [path_lib '\help\',mskblk,'.pdf'];
      | eval('open(doc_path)');
      mask TypeOptions OutputFixedPointDatatype: uint8 | int8 | uint16 | int16 | uint32 | int32
      mask Display:
      | dispmin=num2str(Min);
      | dispmax=num2str(Max);
      | TofxpLib_mask = ['To FXP \n ' 'Resolution (Physical) = ' num2str(Resol) '\n Offset (Physical) =' num2str(Offset) '\n Range (Physical) =' dispmin ' / ' ,dispmax];
      | disp(TofxpLib_mask);
      | port_label('input',1,'phys')
      | port_label('output',1,'fxp')
      | plot([5,5,5])
      | plot([6,6,6])
  AEMS_FXP_TO_FLOAT : Subsystem  Tag=[LIB]  mask(AEMS_FXP_TO_FLOAT){Resol=0.5, Offset=0}
      mask prompts: Resol "Resolution (Physical)"; Offset "Offset (Physical)"
      mask help: Converts the fixed point value into floating point value.
      settings: AttributesFormatString=|
      | %<MaskType>
      | Resolution = %<Resol>
      | Offset = %<Offset>
      mask Help:
      | eval('path_lib=fileparts(which(''AEMS_Standard_Library''));');
      | mskblk=get_param(gcbh,'MaskType');
      | doc_path = [path_lib '\help\',mskblk,'.pdf'];
      | eval('open(doc_path)');
      mask Display:
      | TofxpLib_mask = ['To PHYS \n ' 'Resolution (Physical) = ' num2str(Resol) '\n Offset (Physical) =' num2str(Offset) ];
      | disp(TofxpLib_mask);
      | port_label('input',1,'fxp')
      | port_label('output',1,'phys')
      | plot([5,5,5])
      | plot([6,6,6])
  AEMS_RAM_SET_MAX : Subsystem  Tag=[LIB]  mask(AEMS_RAM_SET_MAX){initial_value=0}
      mask prompts: initial_value "Initial Value :"
      mask help:
      | Set RAM (Max)
      |
      | I/O
      |  input
      |    The maximum of this value is assigned to "max_value."
      |
      |  start
      |    1 : Compute "max_value."
      |    0 : Hold
      |
      |  clear
      |    1 : Initialize "max_value" to the initial value.
      |    0 : None
      |
      |  max_value
      |    The maximum value of "input."
      mask init:
      | name=get_param(gcb,'MaskValueString');
      | initial_value=str2num(name);
      settings: AttributesFormatString=%<MaskType>
      mask Help:
      | eval('path_lib=fileparts(which(''AEMS_Standard_Library''));');
      | mskblk=get_param(gcbh,'MaskType');
      | doc_path = [path_lib '\help\',mskblk,'.pdf'];
      | eval('open(doc_path)');
      mask Display: disp(sprintf('Initial Value = %s', char(name)))
  AEMS_RAM_SET_MIN : Subsystem  Tag=[LIB]  mask(AEMS_RAM_SET_MIN){initilal_value=65535}
      mask prompts: initilal_value "Initial Value :"
      mask help:
      | Set RAM (Min)
      |
      | I/O
      |  input
      |    The minimum of this value is assigned to "min_value."
      |
      |  start
      |    1 : Compute "min_value."
      |    0 : Hold
      |
      |  clear
      |    1 : Initialize "min_value" to the initial value.
      |    0 : None
      |
      |  min_value
      |    The minimum value of "input."
      mask init:
      | name=get_param(gcb,'MaskValueString');
      | initial_value=str2num(name);
      settings: AttributesFormatString=%<MaskType>
      mask Help:
      | eval('path_lib=fileparts(which(''AEMS_Standard_Library''));');
      | mskblk=get_param(gcbh,'MaskType');
      | doc_path = [path_lib '\help\',mskblk,'.pdf'];
      | eval('open(doc_path)');
      mask Display: disp(sprintf('Initial Value = %s', char(name)))
  AEMS_TO_FXP_WITH_LIMIT : Subsystem  Tag=[LIB]  mask(AEMS_TO_FXP_WITH_LIMIT){Resol=1, Offset=0, Min=0, Max=127, OutputFixedPointDatatype=int8}
      mask prompts: Resol "Resolution (physical)"; Offset "Offset (Physical)"; Min "Minimum (Physical)"; Max "Maximum (Physical)"
      mask help: Converts the Floating/Fixed point input into Fixed point value
      mask init:
      | ThisBlk = gcb;
      | Bpath = [ThisBlk,'/OutputDatatype'];
      | OutputDatatype = get_param(gcb,'OutputFixedPointDatatype');
      | set_param(Bpath,'OutDataTypeStr',OutputDatatype);
      | 
      | Min_Hex = (Min-Offset)/Resol; %Hex value of Min
      | Max_Hex = (Max-Offset)/Resol; %Hex value of Max
      | 
      | %Initial Checks:
      | if (Min > Max)
      |     disp(Min);
      |     disp(Max);    
      |     error('Min Value Should be less than the Max value');
      | end
      | 
      | % Possible max_hex > max_hex > min_hex > possible min_hex
      | 
      | %Chk for min/max values
      | 
      | switch OutputDatatype
      |     
      |     case 'int8'
      |         Possible_Min_Hex = -128;
      |         Possible_Max_Hex = 127;
      |     case 'uint8'
      |         Possible_Min_Hex = 0;
      |         Possible_Max_Hex = 255;
      |     case 'int16'
      |         Possible_Min_Hex = -32768;
      |         Possible_Max_Hex = 32767;
      |     case 'uint16'
      |         Possible_Min_Hex = 0;
      |         Possible_Max_Hex = 65535;
      |     case 'int32'
      |         Possible_Min_Hex = -2147483648;
      |         Possible_Max_Hex = 2147483647;
      |     case 'uint32'
      |         Possible_Min_Hex = 0;
      |         Possible_Max_Hex = 4294967295;
      | 
      | end
      | 
      | if (Min_Hex < Possible_Min_Hex)
      |     %     msg = sprintf(['\n','For the resolution of "',num2str(Resol),'" and Offset of "',num2str(Offset),'",\n',...
      |     %         'and output dataThe Physical Max value "',num2str(Max) ,'" can''t fit in 2 byte']);
      |     msg = sprintf(['\n','The physical min "',num2str(Min),'" is invalid for the specified configuration,\n',...
      |         ' Resolution = "',num2str(Resol),'",Offset = "',num2str(Offset),'", OutputDataType "',OutputDatatype,'"']);
      |     error(msg); %#ok<SPERR>
      | elseif (Max_Hex > Possible_Max_Hex)
      |     msg = sprintf(['\n','The physical max "',num2str(Max),'" is invalid for the specified configuration,\n',...
      |         ' Resolution = "',num2str(Resol),'",Offset = "',num2str(Offset),'", OutputDataType "',OutputDatatype,'"']);
      |     error(msg); %#ok<SPERR>
      | end
      settings: AttributesFormatString=%<MaskType>\nResolution (physical) = %<Resol>\nOffset (Physical) = %<Offset>\nMinimum (Physical) = %<Min>\nMaximum (Physical) = %<Max>\nOutput Fixed Point Datatype=%<OutputFixedPointDatatype>
      mask Help:
      | eval('path_lib=fileparts(which(''AEMS_Standard_Library''));');
      | doc_path = [path_lib '\help\AEMS_TO_FXP_WITH_LIMIT.pdf'];
      | eval('open(doc_path)')
      mask TypeOptions OutputFixedPointDatatype: uint8 | int8 | uint16 | int16 | uint32 | int32
      mask Display:
      | disp('AEMS_TO_FXP_WITH_LIMIT')
      | port_label('input',1,'phys_value')
      | port_label('output',1,'fxp_value')
